simulink library "did"  (R2021b)
settings: Solver=VariableStepAuto  StartTime=0.0  StopTime=10.0  RelTol=1e-3
undefined symbols (not defined in the file): ADID_DODRange_pct, ADID_SOCRange_pct, ADID_TempRange_C, DiscIntNeverNeededParam, ENUM_CHRGPLUGSTA_AC, ENUM_CHRGPLUGSTA_DC, ENUM_CHRGPLUGSTA_NONE, ENUM_DRIVETRAIN_AWD, ENUM_DRIVETRAIN_FWD, ENUM_DRIVETRAIN_RWD, ENUM_EXTCHRGSTS_CHARGING, ENUM_OBCV2LSTA_WORKING, ENUM_PWRSTASW_READY, ENUM_VEHICLETYPE_D21, ENUM_VEHICLETYPE_D31F25, ENUM_VEHICLETYPE_D31HAWD, ENUM_VEHICLETYPE_D31HRWD, HOUR2SEC, HUNDRED, KDID_CPSAVehSpdThres_kph, KDID_DIDModelVersion_raw, KDID_DoDChrgCycle_s, KDID_FiveKmEquivEnergy_Wh, KDID_FlashInitDIDModelVersion_raw, KDID_IPSAVehSpdThres_kph, KDID_PropActiveTripThres_s, KDID_PSARResetThres_sec, KDID_RESSCNTSDODRNGAXIS_enum, KDID_RESSTIMESOCRNGAXIS_enum, KDID_RESSTTEMPRNGAXIS_enum, KDID_WarnUpPropActiveThres_s, KDID_WarnUpVehOperIdleThres_mph, KDID_WarnUpVehOperIdleThres_s, KDID_WarnUpVehOperThres_mph, KDID_WarnUpVehOperThres_s, KPH2MPH, KXX2XX, MINUSONE_FLOAT, ONE_FLOAT, ONE_INT, ONE_INT16, ONE_PERCENT, TRUE, UINT16_MAX, UINT32_MAX, XX2KXX, ZERO_FLOAT, ZERO_INT, ZERO_INT16, ZERO_INT32
libraries: hcu_lib x112, simulink x10, nmm x1
(part 2 of 4)

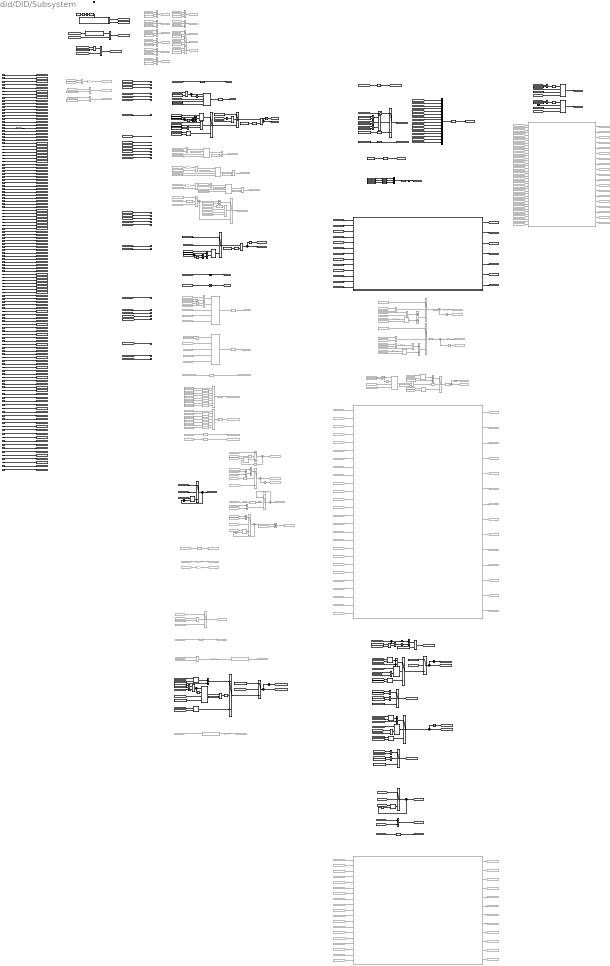
== system did/DID/Subsystem ==
  note: Flash data selector
  note: Model Version
  note: 0xF810: Protocol Identification
  note: 0xF896: Total Number of Propulsion System Active Events
  note: code_clear ??
  note: 0xF44D: Engine run time while MIL activated
  note: 0xF431: Distance traveled since DTCs cleared
  note: 0xF430: Number of warm-ups since DTCs cleared
  note: add debounce?
  note: 0xF421: Distance Traveled While MIL is Activated
  note: 0xF41F: Time Since Engine Start
  note: 0xF40D: Vehicle Speed Sensor
  note: 0xF449: Accelerator Pedal Position D
  note: 0xF44A: Accelerator Pedal Position E
  note: add debounce?
  note: 0xF44E: Engine run time since DTCs cleared
  note: 0xF45B: Hybrid Battery Pack Remaining Charge
  note: 0xF49A: Hybrid/EV Battery System Voltage
  note: 0xF4D1
  note: 0xF4DA
  note: 0xF4D4
  note: 0xF4B9
  note: 0xF4D6
  note: 0xF4D0
  note: SOH?
  note: 0xF4A6
  note: 0xF4B2
  note: Annex G
  note: Annex B
  note: 0xF802: Vehicle Identification Number
  note: 0xF804: Calibration Identifications
  note: 0xF813: Certification Test Group/Engine Family Number
  note: 0xF80A: ECUNAME
  note: 0xF881: High Voltage Battery Net Amp Hours
  note: 0xF882: Ignition Counter
  note: 0xF88C: Positive Kinetic Energy
  note: 0xF88D: Total Distance Travelled
  task_time_s : Inport
  VTQD_VehActSpd_kph : Inport  Port=2
  VPMM_SysPowerMode_enum : Inport  Port=3
  VPMM_DrivetrainSelect_enum : Inport  Port=4
  VDDM_VehMalfunLevel_enum : Inport  Port=5
  VDDM_LimpHomeAct_flg : Inport  Port=6
  VDDM_EnterNewOperCyc_flg : Inport  Port=7
  VINP_CANMsgValidESC1_flg : Inport  Port=8
  VINP_ODOMETER_km : Inport  Port=9
  VINP_CANMsgValidMETER1_flg : Inport  Port=10
  VINP_ClearDTCcmd_flg : Inport  Port=11
  VDHP_LowIdleAccPedal_flg : Inport  Port=12
  VDHP_EAPS1NRM_pct : Inport  Port=13
  VDHP_EAPS2NRM_pct : Inport  Port=14
  VINP_HVBattSOC_pct : Inport  Port=15
  VINP_HVBattPackVolt_V : Inport  Port=16
  VINP_ExtChrgSta_enum : Inport  Port=17
  VINP_HVBattCurr_A : Inport  Port=18
  VINP_HVBattVolt_V : Inport  Port=19
  VINP_ChrgPlugSta_enum : Inport  Port=20
  VINP_HVBPwrAvailChrg_kW : Inport  Port=21
  VINP_HVBCellVoltMax_mV : Inport  Port=22
  VINP_HVBCellVoltMin_mV : Inport  Port=23
  VINP_HVBSOH_pct : Inport  Port=24
  VINP_CANMsgValidMCUBR1_flg : Inport  Port=25
  VINP_CANMsgValidBMS6_flg : Inport  Port=26
  VINP_CANMsgValidBMS1_flg : Inport  Port=27
  VINP_CANMsgValidCCU2_flg : Inport  Port=28
  VINP_CANMsgValidBMS4_flg : Inport  Port=29
  VINP_CellTempAvg_C : Inport  Port=30
  VINP_OBCV2LSta_enum : Inport  Port=31
  VINP_RrMCUDCBusCurr_A : Inport  Port=32
  VINP_RrMCUDCBusVolt_V : Inport  Port=33
  VINP_FrMCUDCBusCurr_A : Inport  Port=34
  VINP_FrMCUDCBusVolt_V : Inport  Port=35
  VINP_CANMsgValidMCUBF1_flg : Inport  Port=36
  VINP_HVBMTempMax_C : Inport  Port=37
  VINP_HVBMTempMin_C : Inport  Port=38
  VINP_MCUBRRealPwrKwSta_kW : Inport  Port=39
  VINP_MCUBFRealPwrKwSta_kW : Inport  Port=40
  VINP_CANMsgValidBMS3_flg : Inport  Port=41
  VINP_VehicleType_enum : Inport  Port=42
  VINP_CarModel1_cnt : Inport  Port=43
  VINP_CarModel2_cnt : Inport  Port=44
  VINP_CarModel3_cnt : Inport  Port=45
  VINP_ECU1_cnt : Inport  Port=46
  VINP_ECU2_cnt : Inport  Port=47
  VINP_Major1_cnt : Inport  Port=48
  VINP_Major2_cnt : Inport  Port=49
  VINP_Minor1_cnt : Inport  Port=50
  VINP_Minor2_cnt : Inport  Port=51
  VINP_Patch1_cnt : Inport  Port=52
  VINP_Patch2_cnt : Inport  Port=53
  VINP_Country1_cnt : Inport  Port=54
  VINP_Country2_cnt : Inport  Port=55
  VINP_Variation_cnt : Inport  Port=56
  VINP_ECUGen1_cnt : Inport  Port=57
  VINP_ECUGen2_cnt : Inport  Port=58
  VINP_FlashMILDIST_km : Inport  Port=59
  VINP_FlashWARMUPS_cnt : Inport  Port=60
  VINP_FlashDelayCLRDIST_km : Inport  Port=61
  VINP_FlashMILTime_min : Inport  Port=62
  VINP_FlashCLRTime_min : Inport  Port=63
  VINP_FlashNUMPSATRIPSFLTMEMCLR_cnt : Inport  Port=64
  VINP_FlashPSAR_sec : Inport  Port=65
  VINP_FlashPSAL_sec : Inport  Port=66
  VINP_FlashIPSAR_sec : Inport  Port=67
  VINP_FlashIPSAL_sec : Inport  Port=68
  VINP_FlashCPSAR_sec : Inport  Port=69
  VINP_FlashCPSAL_sec : Inport  Port=70
  VINP_FlashHVBNAH_Ah : Inport  Port=71
  VINP_FlashIGNCNTR_cnt : Inport  Port=72
  VINP_FlashTNBCPSAR_Ahr : Inport  Port=73
  VINP_FlashTNBCPSAL_Ahr : Inport  Port=74
  VINP_FlashTNECPSAR_kWh : Inport  Port=75
  VINP_FlashTNECPSAL_kWh : Inport  Port=76
  VINP_FlashTEBPSAR_kWh : Inport  Port=77
  VINP_FlashTEBPSAL_kWh : Inport  Port=78
  VINP_FlashTGEOVCR_kWh : Inport  Port=79
  VINP_FlashTGEOVCL_kWh : Inport  Port=80
  VINP_FlashGECHGOVCDCR_kWh : Inport  Port=81
  VINP_FlashGECHGOVCDCL_kWh : Inport  Port=82
  VINP_FlashGECHGOVCACR_kWh : Inport  Port=83
  VINP_FlashGECHGOVCACL_kWh : Inport  Port=84
  VINP_FlashRESSV2XENNONPSAR_kWh : Inport  Port=85
  VINP_FlashRESSV2XENNONPSAL_kWh : Inport  Port=86
  VINP_FlashODOMETER_km : Inport  Port=87
  VINP_FlashPKERNumerator_kphsqr : Inport  Port=88
  VINP_FlashPKELNumerator_kphsqr : Inport  Port=89
  VINP_FlashResetCDEODTR_km : Inport  Port=90
  VINP_FlashTempPSAR_sec : Inport  Port=91
  VINP_FlashAvgBattTempPSAR_C : Inport  Port=92
  VINP_FlashTempPSAL_sec : Inport  Port=93
  VINP_FlashAvgBattTempPSAL_C : Inport  Port=94
  VINP_FlashOVCR_sec : Inport  Port=95
  VINP_FlashAvgBattTempOVCR_C : Inport  Port=96
  VINP_FlashOVCL_sec : Inport  Port=97
  VINP_FlashAvgBattTempOVCL_C : Inport  Port=98
  VINP_FlashOFFR_sec : Inport  Port=99
  VINP_FlashAvgBattTempOFFR_C : Inport  Port=100
  VINP_FlashOFFL_sec : Inport  Port=101
  VINP_FlashAvgBattTempOFFL_C : Inport  Port=102
  VINP_FlashHVBNE_kWh : Inport  Port=103
  VINP_FlashQTYPSATRIPSR_cnt : Inport  Port=104
  VINP_FlashQTYPSATRIPSL_cnt : Inport  Port=105
  VINP_FlashRESSCNTDODRNGR_cnt : Inport  Port=106
  VINP_FlashETMBTOER_kWh : Inport  Port=107
  VINP_FlashETMBTOEL_kWh : Inport  Port=108
  VINP_FlashRESSCNTDODRNGL_cnt : Inport  Port=109
  VINP_FlashETMATOER_kWh : Inport  Port=110
  VINP_FlashETMATOEL_kWh : Inport  Port=111
  VINP_FlashRESSTIMESOCPSARNGR_s : Inport  Port=112
  VINP_FlashRESSTIMESOCPSARNGL_s : Inport  Port=113
  VINP_FlashRESSTIMESOCCHGRNGR_s : Inport  Port=114
  VINP_FlashRESSTIMESOCOFFRNGL_s : Inport  Port=115
  VINP_FlashMAXBATTEMPL_C : Inport  Port=116
  VINP_FlashMINBATTEMPL_C : Inport  Port=117
  VINP_FlashRESSTIMESOCCHGRNGL_s : Inport  Port=118
  VINP_FlashRESSTIMESOCOFFRNGR_s : Inport  Port=119
  VINP_FlashAVGBATTEMPL_sec : Inport  Port=120
  VINP_FlashAVGBATTEMPL_C : Inport  Port=121
  VINP_VinCode_cnt : Inport  Port=122
  VINP_FlashModelVersion_raw : Inport  Port=123
  VINP_FlashModelVersionChksum_raw : Inport  Port=124
  Enable : EnablePort
  0xF819: Total Propulsion System Active Time : Subsystem
  0xF885 - 0xF88B : Subsystem  Commented=on
  0xF88E - 0xF890 : Subsystem  Commented=on
  0xF898-0xF8 : Subsystem  Commented=on
  1-D Lookup Table : Lookup_n-D  NumberOfTableDimensions=1  BreakpointsForDimension1=[ENUM_DRIVETRAIN_RWD;ENUM_DRIVETRAIN_FWD;ENUM_DRIVETRAIN_AWD]  Table=[uint8('R');uint8('F');uint8('A')]  InterpMethod=Nearest  InternalRulePriority=Speed  RndMeth=Simplest  InputSameDT=on
  AND : Logic  Commented=on  AllPortsSameDT=off  OutDataTypeStr=boolean
  AND2 : Logic  AllPortsSameDT=off  OutDataTypeStr=boolean
  AND6 : Logic  AllPortsSameDT=off  OutDataTypeStr=boolean
  Add : Sum
  Add1 : Sum  Commented=on
  Add2 : Sum
  Add3 : Sum
  Add6 : Sum  Commented=on
  Bitwise OR1 : simulink/Logic and Bit Operations/Bitwise Operator  Commented=on  logicop=OR  UseBitMask=off  NumInputPorts=7  BitMask=bin2dec('00000000000000000000')  BitMaskRealWorld=Stored Integer
  Bitwise OR123 : simulink/Logic and Bit Operations/Bitwise Operator  Commented=on  logicop=OR  UseBitMask=off  NumInputPorts=8  BitMask=bin2dec('00000000000000000000')  BitMaskRealWorld=Stored Integer
  Cast To Boolean : DataTypeConversion  OutDataTypeStr=boolean
  Checksum : Subsystem
  Constant{,5,26,28,34} (5 alike) : Constant  Value=ENUM_PWRSTASW_READY
  Constant1 : Constant  Value=UINT32_MAX
  Constant10 : Constant  Commented=on  Value=KDID_WarnUpVehOperThres_s
  Constant{32,59,65..68,105} (7 alike) : Constant  Commented=on  Value=ZERO_FLOAT
  Constant11 : Constant  Commented=on  Value=KDID_WarnUpVehOperThres_s
  Constant113 : Constant  Value=ZERO_FLOAT
  Constant12 : Constant  Commented=on  Value=KDID_WarnUpVehOperIdleThres_s
  Constant13 : Constant  Commented=on  Value=KDID_WarnUpVehOperIdleThres_s
  Constant14 : Constant  Commented=on  Value=KDID_WarnUpVehOperIdleThres_mph
  Constant{15,42,44..45,47..48,51..54,57..58,61..63,69..77} (24 alike) : Constant  Commented=on  Value=ZERO_INT
  Constant16 : Constant  Value=ZERO_FLOAT
  Constant17 : Constant  Value=UINT16_MAX
  Constant{6,18..19,25} (4 alike) : Constant  Commented=on  Value=ENUM_PWRSTASW_READY
  Constant2 : Constant  Commented=on  Value=ONE_INT
  Constant20 : Constant  Commented=on  Value=UINT16_MAX
  Constant21 : Constant  Value=ZERO_INT32
  Constant22 : Constant  Value=ONE_PERCENT  OutDataTypeStr=single
  Constant23 : Constant  Value=ZERO_INT16
  Constant24 : Constant  Commented=on  Value=UINT16_MAX
  Constant27 : Constant  Value=ONE_INT16
  Constant29 : Constant  Value=KDID_PropActiveTripThres_s
  Constant3 : Constant  Value=ZERO_FLOAT
  Constant30 : Constant  Value=KDID_PropActiveTripThres_s
  Constant31 : Constant  Commented=on  Value=ENUM_EXTCHRGSTS_CHARGING
  Constant33 : Constant  Value=UINT32_MAX
  Constant35 : Constant  Value=UINT32_MAX
  Constant36 : Constant  Value=ONE_INT
  Constant37 : Constant  Value=ZERO_FLOAT  OutDataTypeStr=uint16
  Constant38 : Constant  Commented=on  Value=KDID_PropActiveTripThres_s
  Constant39 : Constant  Value=ENUM_DRIVETRAIN_RWD
  Constant4 : Constant  Value=UINT16_MAX
  Constant40 : Constant  Value=ENUM_DRIVETRAIN_RWD
  Constant41 : Constant  Value=ENUM_DRIVETRAIN_RWD
  Constant43 : Constant  Commented=on  Value=ONE_INT
  Constant46 : Constant  Value=ONE_PERCENT  OutDataTypeStr=single
  Constant49 : Constant  Commented=on  Value=KDID_PropActiveTripThres_s
  Constant50 : Constant  Value=ZERO_FLOAT  OutDataTypeStr=single
  Constant55 : Constant  Value=KDID_FlashInitDIDModelVersion_raw
  Constant56 : Constant  Value=ZERO_FLOAT  OutDataTypeStr=single
  Constant60 : Constant  Value=ONE_FLOAT
  Constant64 : Constant  Value=TRUE
  Constant7 : Constant  Commented=on  Value=KDID_WarnUpPropActiveThres_s
  Constant79 : Constant  Commented=on  Value=ONE_INT16
  Constant8 : Constant  Commented=on  Value=KDID_WarnUpPropActiveThres_s
  Constant9 : Constant  Commented=on  Value=KDID_WarnUpVehOperThres_mph
  Data Type Conversion : DataTypeConversion  OutDataTypeStr=single
  Data Type Conversion1 : DataTypeConversion  OutDataTypeStr=uint16
  Data Type Conversion10 : DataTypeConversion  Commented=on  OutDataTypeStr=uint16
  Data Type Conversion{4..5,11,14} (4 alike) : DataTypeConversion  OutDataTypeStr=uint8
  Data Type Conversion{6..8,12,15} (5 alike) : DataTypeConversion  Commented=on
  Data Type Conversion13 : DataTypeConversion
  Data Type Conversion16 : DataTypeConversion  Commented=on  OutDataTypeStr=uint8
  Data Type Conversion17 : DataTypeConversion  Commented=on  OutDataTypeStr=uint8
  Data Type Conversion2 : DataTypeConversion  OutDataTypeStr=single
  Data Type Conversion23 : DataTypeConversion  Commented=on  OutDataTypeStr=single
  Data Type Conversion25 : DataTypeConversion  Commented=on  OutDataTypeStr=single
  Data Type Conversion29 : DataTypeConversion  Commented=on  OutDataTypeStr=uint16
  Data Type Conversion3 : DataTypeConversion  OutDataTypeStr=single
  Data Type Conversion9 : DataTypeConversion  Commented=on  OutDataTypeStr=uint16
  Delay : Delay  DelayLengthSource=Input port  DelayLengthUpperLimit=255
      settings: InputPortMap=u0,p1
  Delay1 : Delay
  Delay2 : Delay  Commented=on  DelayLength=1
  Detect Decrease : simulink/Logic and Bit Operations/Detect Decrease  Commented=on  vinit=0.0  OutDataTypeStr=boolean
  Detect Increase : simulink/Logic and Bit Operations/Detect Increase  vinit=0.0  OutDataTypeStr=boolean
  Detect Increase1 : simulink/Logic and Bit Operations/Detect Increase  vinit=0.0  OutDataTypeStr=boolean
  Detect Increase2 : simulink/Logic and Bit Operations/Detect Increase  Commented=on  vinit=0.0  OutDataTypeStr=boolean
  Detect Increase3 : simulink/Logic and Bit Operations/Detect Increase  vinit=0.0  OutDataTypeStr=boolean
  Detect Increase4 : simulink/Logic and Bit Operations/Detect Increase  Commented=on  vinit=0.0  OutDataTypeStr=boolean
  Detect Increase5 : simulink/Logic and Bit Operations/Detect Increase  Commented=on  vinit=0.0  OutDataTypeStr=boolean
  Divide : Product  Inputs=*/
  Divide1 : Product  Inputs=*/
  Divide2 : Product  Inputs=*/
  Equal{,2,9,13,15..17,21..22} (9 alike) : RelationalOperator  Operator===  OutDataTypeStr=boolean  RndMeth=Simplest
  Equal{1,8,10,12,18} (5 alike) : RelationalOperator  Commented=on  Operator===  OutDataTypeStr=boolean  RndMeth=Simplest
  Equal11 : RelationalOperator  OutDataTypeStr=boolean  RndMeth=Simplest
  Equal{3..5,7,14} (5 alike) : RelationalOperator  Commented=on  OutDataTypeStr=boolean  RndMeth=Simplest
  Equal19 : RelationalOperator  Operator=>  OutDataTypeStr=boolean  RndMeth=Simplest
  Equal20 : RelationalOperator  Operator=>  OutDataTypeStr=boolean  RndMeth=Simplest
  Equal23 : RelationalOperator  OutDataTypeStr=boolean  RndMeth=Simplest
  Equal6 : RelationalOperator  Commented=on  Operator=<=  OutDataTypeStr=boolean  RndMeth=Simplest
  From100 : From  Commented=on  GotoTag=VINP_FlashRESSV2XENNONPSAR_kWh
  From101 : From  Commented=on  GotoTag=VINP_FlashRESSV2XENNONPSAL_kWh
  From102 : From  Commented=on  GotoTag=VINP_CANMsgValidCCU2_flg
  From103 : From  Commented=on  GotoTag=VINP_ChrgPlugSta_enum
  From{15,17,20,31,35,75,106,158..159,162,246} (11 alike) : From  Commented=on  GotoTag=task_time_s
  From107 : From  Commented=on  GotoTag=VINP_CellTempAvg_C
  From108 : From  Commented=on  GotoTag=VINP_FlashTempPSAR_sec
  From110 : From  Commented=on  GotoTag=VDID_FlashAvgBattTempPSAR_C
  From111 : From  Commented=on  GotoTag=VINP_FlashTempPSAL_sec
  From112 : From  Commented=on  GotoTag=VDID_FlashAvgBattTempPSAL_C
  From113 : From  Commented=on  GotoTag=VINP_FlashOVCR_sec
  From116 : From  Commented=on  GotoTag=VDID_FlashAvgBattTempOVCR_C
  From117 : From  Commented=on  GotoTag=VINP_FlashOVCL_sec
  From125 : From  Commented=on  GotoTag=VDID_FlashAvgBattTempOVCL_C
  From129 : From  Commented=on  GotoTag=VINP_FlashOFFR_sec
  From131 : From  Commented=on  GotoTag=VDID_FlashAvgBattTempOFFR_C
  From132 : From  Commented=on  GotoTag=VINP_FlashOFFL_sec
  From133 : From  Commented=on  GotoTag=VDID_FlashAvgBattTempOFFL_C
  From{14,30,60,76,96,134,261} (7 alike) : From  Commented=on  GotoTag=VPMM_SysPowerMode_enum
  From135 : From  Commented=on  GotoTag=VDID_HVBattPwr_kW
  From136 : From  Commented=on  GotoTag=VINP_CANMsgValidBMS4_flg
  From140 : From  Commented=on  GotoTag=VINP_CANMsgValidBMS6_flg
  From141 : From  Commented=on  GotoTag=VDID_FlashHVBNAH_Ah
  From142 : From  Commented=on  GotoTag=VDID_NoteAResetCondition_flg
  From152 : From  Commented=on  GotoTag=VDID_DelayHVBNAH_As
  From153 : From  Commented=on  GotoTag=VINP_DIDResetNetAhrs_flg
  From{41,46,74,154,160,272,325} (7 alike) : From  Commented=on  GotoTag=VDID_HVBattCurr_A
  From155 : From  Commented=on  GotoTag=VINP_DIDResetNetAhrs_flg
  From{24,34,37..38,79,156..157,208} (8 alike) : From  Commented=on  GotoTag=VINP_ClearDTCcmd_flg
  From16 : From  Commented=on  GotoTag=VTQD_VehActSpd_kph
  From{40,48,161,273} (4 alike) : From  Commented=on  GotoTag=VINP_HVBattVolt_V
  From163 : From  Commented=on  GotoTag=VDID_FlashHVBNE_kWh
  From164 : From  Commented=on  GotoTag=VDID_DelayHVBNE_kWs
  From177 : From  Commented=on  GotoTag=VDID_DelayIGNCNTR_cnt
  From178 : From  Commented=on  GotoTag=VINP_FlashIGNCNTR_cnt
  From179 : From  Commented=on  GotoTag=VDID_DelayIGNCNTR_cnt
  From18 : From  Commented=on  GotoTag=VDHP_LowIdleAccPedal_flg
  From180 : From  Commented=on  GotoTag=VINP_FlashIGNCNTR_cnt
  From19 : From  Commented=on  GotoTag=VTQD_VehActSpd_kph
  From21 : From  Commented=on  GotoTag=KDID_WarnUpPropActive_flg
  From22 : From  Commented=on  GotoTag=KDID_WarnUpVehOper_flg
  From222 : From  Commented=on  GotoTag=VINP_OBCV2LSta_enum
  From23 : From  Commented=on  GotoTag=KDID_WarnUpVehOperIdle_flg
  From245 : From  Commented=on  GotoTag=VDID_HVBattPwr_kW
  From247 : From  Commented=on  GotoTag=VINP_CANMsgValidBMS1_flg
  From248 : From  Commented=on  GotoTag=VDID_NoteAResetCondition_flg
  From249 : From  Commented=on  GotoTag=VINP_FlashRESSCNTDODRNGR_cnt
  From250 : From  Commented=on  GotoTag=VINP_FlashRESSCNTDODRNGL_cnt
  From251 : From  Commented=on  GotoTag=VINP_RrMCUDCBusCurr_A
  From252 : From  Commented=on  GotoTag=VINP_RrMCUDCBusVolt_V
  From253 : From  Commented=on  GotoTag=VINP_FlashETMATOER_kWh
  From254 : From  Commented=on  GotoTag=VINP_FlashETMATOEL_kWh
  From255 : From  Commented=on  GotoTag=VINP_CANMsgValidMCUBR1_flg
  From256 : From  Commented=on  GotoTag=VINP_FrMCUDCBusCurr_A
  From257 : From  Commented=on  GotoTag=VINP_FrMCUDCBusVolt_V
  From258 : From  Commented=on  GotoTag=VINP_FlashETMBTOER_kWh
  From259 : From  Commented=on  GotoTag=VINP_FlashETMBTOEL_kWh
  From260 : From  Commented=on  GotoTag=VINP_CANMsgValidMCUBF1_flg
  From262 : From  Commented=on  GotoTag=VINP_ChrgPlugSta_enum
  From263 : From  Commented=on  GotoTag=VINP_CANMsgValidBMS6_flg
  From264 : From  Commented=on  GotoTag=VINP_HVBattSOC_pct
  From265 : From  Commented=on  GotoTag=VINP_FlashRESSTIMESOCPSARNGR_s
  From266 : From  Commented=on  GotoTag=VINP_FlashRESSTIMESOCPSARNGL_s
  From267 : From  Commented=on  GotoTag=VINP_ExtChrgSta_enum
  From268 : From  Commented=on  GotoTag=VINP_FlashRESSTIMESOCCHGRNGR_s
  From269 : From  Commented=on  GotoTag=VINP_FlashRESSTIMESOCCHGRNGL_s
  From270 : From  Commented=on  GotoTag=VINP_FlashRESSTIMESOCOFFRNGR_s
  From271 : From  Commented=on  GotoTag=VINP_FlashRESSTIMESOCOFFRNGL_s
  From274 : From  Commented=on  GotoTag=VDID_HVBattPwr_kW
  From275 : From  Commented=on  GotoTag=VDID_FlashMAXBATTEMPL_C
  From276 : From  Commented=on  GotoTag=VINP_HVBMTempMax_C
  From{277,370,375,379..380} (5 alike) : From  Commented=on  GotoTag=VINP_CANMsgValidMETER1_flg
  From278 : From  Commented=on  GotoTag=VDID_FlashMINBATTEMPL_C
  From279 : From  Commented=on  GotoTag=VINP_HVBMTempMin_C
  From280 : From  Commented=on  GotoTag=VINP_CANMsgValidBMS4_flg
  From281 : From  Commented=on  GotoTag=VINP_FlashAVGBATTEMPL_sec
  From282 : From  Commented=on  GotoTag=VDID_FlashAVGBATTEMPL_C
  From283 : From  Commented=on  GotoTag=VINP_CellTempAvg_C
  From285 : From  Commented=on  GotoTag=VDID_HVBattPwrDischrg_kW
  From286 : From  Commented=on  GotoTag=VINP_MCUBRRealPwrKwSta_kW
  From287 : From  Commented=on  GotoTag=VINP_MCUBFRealPwrKwSta_kW
  From288 : From  Commented=on  GotoTag=VINP_CANMsgValidBMS3_flg
  From3 : From  Commented=on  GotoTag=VDDM_EnterNewOperCyc_flg
  From32 : From  Commented=on  GotoTag=VDDM_LimpHomeActTmp_flg
  From33 : From  Commented=on  GotoTag=VDDM_LimpHomeAct_flg
  From{335,337,339..343,345,354..356} (11 alike) : From  Commented=on  GotoTag=VDID_FlashValid_flg
  From336 : From  Commented=on  GotoTag=VINP_FlashHVBNAH_Ah
  From338 : From  Commented=on  GotoTag=VINP_FlashHVBNE_kWh
  From344 : From  Commented=on  GotoTag=VINP_FlashAvgBattTempPSAL_C
  From346 : From  Commented=on  GotoTag=VINP_FlashAvgBattTempOVCR_C
  From347 : From  Commented=on  GotoTag=VINP_FlashAvgBattTempOVCL_C
  From348 : From  Commented=on  GotoTag=VINP_FlashAvgBattTempOFFR_C
  From349 : From  Commented=on  GotoTag=VINP_FlashAvgBattTempPSAR_C
  From350 : From  Commented=on  GotoTag=VINP_FlashAvgBattTempOFFL_C
  From351 : From  Commented=on  GotoTag=VINP_FlashMAXBATTEMPL_C
  From352 : From  Commented=on  GotoTag=VINP_FlashMINBATTEMPL_C
  From353 : From  Commented=on  GotoTag=VINP_FlashAVGBATTEMPL_C
  From{357,368,371,373,381} (5 alike) : From  Commented=on  GotoTag=VINP_ODOMETER_km
  From367 : From  Commented=on  GotoTag=VINP_FlashODOMETER_km
  From369 : From  Commented=on  GotoTag=VINP_FlashODOMETER_km
  From372 : From  Commented=on  GotoTag=VDID_ODOMETERLostConn_km
  From374 : From  Commented=on  GotoTag=VDID_ODOMETERLostDelay_km
  From376 : From  Commented=on  GotoTag=VDID_ODOMETERLostDelay_km
  From377 : From  Commented=on  GotoTag=VDID_ODOMETERLost_km
  From378 : From  Commented=on  GotoTag=VINP_FlashODOMETERLost_km
  From39 : From  Commented=on  GotoTag=VINP_HVBattSOC_pct
  From51 : From  Commented=on  GotoTag=VDID_HVBattPwrChrg_kW
  From52 : From  Commented=on  GotoTag=VINP_HVBPwrAvailChrg_kW
  From54 : From  Commented=on  GotoTag=VINP_HVBSOH_pct
  From55 : From  Commented=on  GotoTag=VINP_HVBCellVoltMax_mV
  From56 : From  Commented=on  GotoTag=VINP_HVBCellVoltMin_mV
  From61 : From  Commented=on  GotoTag=VINP_ExtChrgSta_enum
  From77 : From  Commented=on  GotoTag=VINP_FlashTNBCPSAR_Ahr
  From78 : From  Commented=on  GotoTag=VINP_FlashMILTime_min
  From8 : From  Commented=on  GotoTag=VINP_FlashWARMUPS_cnt
  From80 : From  Commented=on  GotoTag=VINP_FlashCLRTime_min
  From81 : From  Commented=on  GotoTag=VINP_CANMsgValidBMS1_flg
  From82 : From  Commented=on  GotoTag=VDID_NoteAResetCondition_flg
  From83 : From  Commented=on  GotoTag=VINP_FlashTNBCPSAL_Ahr
  From84 : From  Commented=on  GotoTag=VDID_HVBattPwrDischrg_kW
  From85 : From  Commented=on  GotoTag=VINP_FlashTNECPSAR_kWh
  From86 : From  Commented=on  GotoTag=VINP_FlashTNECPSAL_kWh
  From87 : From  Commented=on  GotoTag=VDID_HVBattPwrChrg_kW
  From88 : From  Commented=on  GotoTag=VINP_ChrgPlugSta_enum
  From89 : From  Commented=on  GotoTag=VINP_FlashTEBPSAR_kWh
  From90 : From  Commented=on  GotoTag=VINP_CANMsgValidBMS6_flg
  From91 : From  Commented=on  GotoTag=VINP_FlashTEBPSAL_kWh
  From92 : From  Commented=on  GotoTag=VINP_ExtChrgSta_enum
  From93 : From  Commented=on  GotoTag=VINP_FlashTGEOVCR_kWh
  From94 : From  Commented=on  GotoTag=VINP_FlashTGEOVCL_kWh
  From95 : From  Commented=on  GotoTag=VINP_FlashGECHGOVCDCR_kWh
  From97 : From  Commented=on  GotoTag=VINP_FlashGECHGOVCDCL_kWh
  From98 : From  Commented=on  GotoTag=VINP_FlashGECHGOVCACR_kWh
  From99 : From  Commented=on  GotoTag=VINP_FlashGECHGOVCACL_kWh
  Gain : Gain  Commented=on  Gain=KPH2MPH
  Gain1 : Gain  Commented=on  Gain=KPH2MPH
  Gain{2..3,14,20} (4 alike) : Gain  Commented=on  Gain=1/HOUR2SEC
  Gain19 : Gain  Gain=MINUSONE_FLOAT
  Gain21 : Gain  Commented=on  Gain=HOUR2SEC
  Gain{5..6,8,27} (4 alike) : Gain  Commented=on  Gain=XX2KXX
  Gain7 : Gain  Commented=on  Gain=HOUR2SEC
  Goto103 : Goto  Commented=on  GotoTag=VDID_HVBNE_kWh
  Goto12 : Goto  Commented=on  GotoTag=KDID_WarnUpPropActive_flg
  Goto13 : Goto  Commented=on  GotoTag=KDID_WarnUpVehOper_flg
  Goto135 : Goto  Commented=on  GotoTag=VDID_MILTIME_min
  Goto136 : Goto  Commented=on  GotoTag=VDID_CLRTIME_min
  Goto137 : Goto  Commented=on  GotoTag=VDID_BATSOC_pct
  Goto138 : Goto  Commented=on  GotoTag=VDID_HEVBATT_V
  Goto139 : Goto  Commented=on  GotoTag=VDID_IGNCNTR_cnt
  Goto14 : Goto  Commented=on  GotoTag=VDID_WARMUPS_cnt
  Goto140 : Goto  Commented=on  GotoTag=VDID_FlashHVBNAH_Ah
  Goto15 : Goto  Commented=on  GotoTag=KDID_WarnUpVehOperIdle_flg
  Goto153 : Goto  Commented=on  GotoTag=VDID_RESSCNTDODRNGR_cnt
  Goto154 : Goto  Commented=on  GotoTag=VDID_RESSCNTDODRNGL_cnt
  Goto155 : Goto  Commented=on  GotoTag=VDID_ETMATOER_kWh
  Goto156 : Goto  Commented=on  GotoTag=VDID_ETMATOEL_kWh
  Goto157 : Goto  Commented=on  GotoTag=VDID_ETMBTOER_kWh
  Goto158 : Goto  Commented=on  GotoTag=VDID_ETMBTOEL_kWh
  Goto159 : Goto  Commented=on  GotoTag=VDID_RESSTIMESOCPSARNGR_s
  Goto160 : Goto  Commented=on  GotoTag=VDID_RESSTIMESOCPSARNGL_s
  Goto161 : Goto  Commented=on  GotoTag=VDID_RESSTIMESOCCHGRNGR_s
  Goto162 : Goto  Commented=on  GotoTag=VDID_RESSTIMESOCCHGRNGL_s
  Goto163 : Goto  Commented=on  GotoTag=VDID_RESSTIMESOCOFFRNGR_s
  Goto164 : Goto  Commented=on  GotoTag=VDID_RESSTIMESOCOFFRNGL_s
  Goto165 : Goto  Commented=on  GotoTag=VDID_MAXBATTEMPL_C
  Goto166 : Goto  Commented=on  GotoTag=VDID_MINBATTEMPL_C
  Goto167 : Goto  Commented=on  GotoTag=VDID_AVGBATTEMPL_C
  Goto176 : Goto  Commented=on  GotoTag=VDID_RESSTTEMPRNGAXIS_enum
  Goto182 : Goto  Commented=on  GotoTag=VDID_RESSTIMESOCRNGAXIS_enum
  Goto183 : Goto  Commented=on  GotoTag=VDID_RESSCNTSDODRNGAXIS_enum
  Goto215 : Goto  Commented=on  GotoTag=VDID_AVGBATTEMPL_sec
  Goto216 : Goto  Commented=on  GotoTag=VDID_BattTempPSAR_sec
  Goto217 : Goto  Commented=on  GotoTag=VDID_BattTempPSAL_sec
  Goto218 : Goto  Commented=on  GotoTag=VDID_OVCR_sec
  Goto219 : Goto  Commented=on  GotoTag=VDID_OVCL_sec
  Goto22 : Goto  Commented=on  GotoTag=VDID_HVBattCurr_Ahps
  Goto220 : Goto  Commented=on  GotoTag=VDID_OFFR_sec
  Goto221 : Goto  Commented=on  GotoTag=VDID_OFFL_sec
  Goto227 : Goto  Commented=on  GotoTag=VDID_HVBATT_A
  Goto228 : Goto  Commented=on  GotoTag=VDID_HEVMODE_enum
  Goto229 : Goto  Commented=on  GotoTag=VDID_STASUP_enum
  Goto237 : Goto  Commented=on  GotoTag=VDID_FlashHVBNE_kWh
  Goto238 : Goto  Commented=on  GotoTag=VDID_FlashAvgBattTempPSAR_C
  Goto239 : Goto  Commented=on  GotoTag=VDID_FlashAvgBattTempPSAL_C
  Goto24 : Goto  Commented=on  GotoTag=VDID_HVESSENER_Whps
  Goto240 : Goto  Commented=on  GotoTag=VDID_FlashAvgBattTempOVCR_C
  Goto241 : Goto  Commented=on  GotoTag=VDID_FlashAvgBattTempOVCL_C
  Goto242 : Goto  Commented=on  GotoTag=VDID_FlashAvgBattTempOFFR_C
  Goto243 : Goto  Commented=on  GotoTag=VDID_FlashAvgBattTempOFFL_C
  Goto244 : Goto  Commented=on  GotoTag=VDID_FlashMAXBATTEMPL_C
  Goto245 : Goto  Commented=on  GotoTag=VDID_FlashMINBATTEMPL_C
  Goto246 : Goto  Commented=on  GotoTag=VDID_FlashAVGBATTEMPL_C
  Goto247 : Goto  Commented=on  GotoTag=VDID_ODOMETERLostConn_km
  Goto248 : Goto  Commented=on  GotoTag=VDID_ODOMETERLost_km
  Goto249 : Goto  Commented=on  GotoTag=VDID_ODOMETERLostDelay_km
  Goto25 : Goto  Commented=on  GotoTag=VDID_HVESSCHARGEACT_kW
  Goto250 : Goto  Commented=on  GotoTag=VDID_ODOMETER_km
  Goto251 : Goto  Commented=on  GotoTag=VINP_FlashODOMETERLost_km
  Goto26 : Goto  Commented=on  GotoTag=VDID_HVESSCHARGELIM_kW
  Goto27 : Goto  Commented=on  GotoTag=VDID_HVBCellVoltMax_V
  Goto29 : Goto  Commented=on  GotoTag=VDID_BATSOH_pct
  Goto30 : Goto  Commented=on  GotoTag=VDID_HVBCellVoltMin_V
  Goto50 : Goto  Commented=on  GotoTag=VDID_TNBCPSAR_Ahr
  Goto53 : Goto  Commented=on  GotoTag=VDID_TNBCPSAL_Ahr
  Goto54 : Goto  Commented=on  GotoTag=VDID_TNECPSAR_kWh
  Goto57 : Goto  Commented=on  GotoTag=VDID_TNECPSAL_kWh
  Goto58 : Goto  Commented=on  GotoTag=VDID_TEBPSAR_kWh
  Goto59 : Goto  Commented=on  GotoTag=VDID_TEBPSAL_kWh
  Goto60 : Goto  Commented=on  GotoTag=VDID_TGEOVCR_kWh
  Goto61 : Goto  Commented=on  GotoTag=VDID_TGEOVCL_kWh
  Goto62 : Goto  Commented=on  GotoTag=VDID_GECHGOVCDCR_kWh
  Goto63 : Goto  Commented=on  GotoTag=VDID_GECHGOVCDCL_kWh
  Goto64 : Goto  Commented=on  GotoTag=VDID_GECHGOVCACR_kWh
  Goto65 : Goto  Commented=on  GotoTag=VDID_GECHGOVCACL_kWh
  Goto66 : Goto  Commented=on  GotoTag=VDID_DelayIGNCNTR_cnt
  Goto67 : Goto  Commented=on  GotoTag=VDID_DelayHVBNAH_As
  Goto69 : Goto  Commented=on  GotoTag=VDID_DelayHVBNE_kWs
  Goto72 : Goto  Commented=on  GotoTag=VDID_RESSV2XENNONPSAR_kWh
  Goto73 : Goto  Commented=on  GotoTag=VDID_RESSV2XENNONPSAL_kWh
  Goto74 : Goto  Commented=on  GotoTag=VDID_AvgBattTempPSAR_C
  Goto75 : Goto  Commented=on  GotoTag=VDID_AvgBattTempPSAL_C
  Goto76 : Goto  Commented=on  GotoTag=VDID_AvgBattTempOVCR_C
  Goto77 : Goto  Commented=on  GotoTag=VDID_AvgBattTempOVCL_C
  Goto78 : Goto  Commented=on  GotoTag=VDID_AvgBattTempOFFR_C
  Goto79 : Goto  Commented=on  GotoTag=VDID_AvgBattTempOFFL_C
  Goto80 : Goto  Commented=on  GotoTag=VDID_HVBattPwr_kW
  Goto85 : Goto  Commented=on  GotoTag=VDID_HVBattPwrChrg_kW
  Goto86 : Goto  Commented=on  GotoTag=VDID_HVBattPwrDischrg_kW
  Goto99 : Goto  Commented=on  GotoTag=VDID_HVBNAH_Ahr
  Ground : Ground
  Initial Value{,1..6,34..37} (11 alike) : hcu_lib/Basic_Blocks/Initial Value
  Initial Value{7..12} (6 alike) : hcu_lib/Basic_Blocks/Initial Value  Commented=on
  Initializable_U32counter : hcu_lib/Basic_Blocks/Initializable_U32counter
  Initializable_U32counter1 : hcu_lib/Basic_Blocks/Initializable_U32counter
  Latch : hcu_lib/Basic_Blocks/Latch  Commented=on
  Latch1 : hcu_lib/Basic_Blocks/Latch  Commented=on
  Latch2 : hcu_lib/Basic_Blocks/Latch  Commented=on
  Logical Operator : Logic  Operator=OR  AllPortsSameDT=off  OutDataTypeStr=boolean
  Logical Operator1 : Logic  Inputs=3  AllPortsSameDT=off  OutDataTypeStr=boolean
  Logical Operator2 : Logic  Commented=on  Inputs=4  AllPortsSameDT=off  OutDataTypeStr=boolean
  Logical Operator3 : Logic  Commented=on  AllPortsSameDT=off  OutDataTypeStr=boolean
  Logical Operator4 : Logic  AllPortsSameDT=off  OutDataTypeStr=boolean
  Logical Operator5 : Logic  Commented=on  Operator=OR  AllPortsSameDT=off  OutDataTypeStr=boolean
  Logical Operator6 : Logic  Commented=on  Operator=OR  AllPortsSameDT=off  OutDataTypeStr=boolean
  Logical Operator7 : Logic  Commented=on  Operator=OR  AllPortsSameDT=off  OutDataTypeStr=boolean
  Logical Operator8 : Logic  Operator=NOT  AllPortsSameDT=off  OutDataTypeStr=boolean
  Logical Operator9 : Logic  AllPortsSameDT=off  OutDataTypeStr=boolean
  Max : MinMax  Inputs=2
  Max1 : MinMax  Inputs=2
  Max3 : MinMax  Function=max  Inputs=2
  Min14 : MinMax  Commented=on  Function=max  Inputs=2
  Min15 : MinMax  Commented=on  Inputs=2
  Minus : Sum  Inputs=+-
  Minus1 : Sum  Commented=on
  Minus2 : Sum  Commented=on
  Minus{3..6} (4 alike) : Sum  Commented=on  Inputs=+-
  Minus7 : Sum  Commented=on
  Minutes_Counter : hcu_lib/Basic_Blocks/Minutes_Counter  Commented=on
  Minutes_Counter1 : hcu_lib/Basic_Blocks/Minutes_Counter  Commented=on
  Mux : Mux  Inputs=3
  Mux1 : Mux  Inputs=16
  NOT{,1,3..4} (4 alike) : Logic  Operator=NOT  AllPortsSameDT=off  OutDataTypeStr=boolean
  NOT2 : Logic  Commented=on  Operator=NOT  AllPortsSameDT=off  OutDataTypeStr=boolean
  NOT6 : Logic  Commented=on  Operator=NOT  AllPortsSameDT=off  OutDataTypeStr=boolean
  OR : Logic  Operator=OR  Inputs=3  AllPortsSameDT=off  OutDataTypeStr=boolean
  Product{,1..2,4,27} (5 alike) : Product  Commented=on
  Reshape : Reshape
  Riemann Integral : hcu_lib/Basic_Blocks/Riemann Integral  Commented=on  Ts=0.005  Total_T=1
  Riemann Integral1 : hcu_lib/Basic_Blocks/Riemann Integral  Commented=on  Ts=0.005  Total_T=1
  Saturation : Saturate  UpperLimit=HUNDRED  LowerLimit=ZERO_FLOAT  OutDataTypeStr=single
  Saturation1 : Saturate  UpperLimit=HUNDRED  LowerLimit=ZERO_FLOAT  OutDataTypeStr=single
  Scheduler : Stateflow chart  TreatAsAtomicUnit=on
  Scheduler1 : Stateflow chart  TreatAsAtomicUnit=on
  Seconds_Counter : hcu_lib/Basic_Blocks/Seconds_Counter
  Shift Arithmetic1 : ArithShift  Commented=on  BitShiftNumber=4  BitShiftDirection=Left
  Shift Arithmetic10 : ArithShift  Commented=on  BitShiftNumber=3  BitShiftDirection=Left
  Shift Arithmetic11 : ArithShift  Commented=on  BitShiftNumber=7  BitShiftDirection=Left
  Shift Arithmetic2 : ArithShift  Commented=on  BitShiftNumber=5  BitShiftDirection=Left
  Shift Arithmetic3 : ArithShift  Commented=on  BitShiftNumber=6  BitShiftDirection=Left
  Shift Arithmetic311 : ArithShift  Commented=on  BitShiftNumber=1  BitShiftDirection=Left
  Shift Arithmetic312 : ArithShift  Commented=on  BitShiftNumber=2  BitShiftDirection=Left
  Shift Arithmetic313 : ArithShift  Commented=on  BitShiftNumber=3  BitShiftDirection=Left
  Shift Arithmetic4 : ArithShift  Commented=on  BitShiftNumber=7  BitShiftDirection=Left
  Shift Arithmetic5 : ArithShift  Commented=on  BitShiftNumber=4  BitShiftDirection=Left
  Shift Arithmetic6 : ArithShift  Commented=on  BitShiftNumber=5  BitShiftDirection=Left
  Shift Arithmetic7 : ArithShift  Commented=on  BitShiftNumber=6  BitShiftDirection=Left
  Shift Arithmetic8 : ArithShift  Commented=on  BitShiftNumber=1  BitShiftDirection=Left
  Square : Math  Operator=square  SaturateOnIntegerOverflow=on
  Square1 : Math  Operator=square  SaturateOnIntegerOverflow=on
  String Constant : StringConstant  String="\"EVCM\""
  String Constant1 : StringConstant  String="\"-\""
  String Constant2 : StringConstant  String="\"ElecVehicleCtrl\""
  String Constant3 : StringConstant  String="\"0\""
  String Constant4 : StringConstant  String="\"S\""
  String to ASCII : StringToASCII  OutputVectorSize=4
  String to ASCII1 : StringToASCII  OutputVectorSize=1
  String to ASCII2 : StringToASCII  OutputVectorSize=15
  String to ASCII3 : StringToASCII  OutputVectorSize=1
  String to ASCII4 : StringToASCII  OutputVectorSize=1
  Subsystem : Subsystem
  Subtract : Sum  Inputs=+-
  Subtract1 : Sum  Inputs=+-
  Subtract2 : Sum
  Subtract3 : Sum
  Subtract6 : Sum  Inputs=+-
  Switch{,1,4..7,9,11,16,61} (10 alike) : Switch  Criteria=u2 > Threshold
  Switch10 : Switch  Criteria=u2 ~= 0
      settings: AttributesFormatString=<%<Criteria>>
  Switch12 : Switch  Criteria=u2 ~= 0
      settings: AttributesFormatString=<%<Criteria>>
  Switch{2..3,8,13..15,17..31} (21 alike) : Switch  Commented=on  Criteria=u2 > Threshold
  Switch60 : Switch  Criteria=u2 ~= 0
      settings: AttributesFormatString=<%<Criteria>>
  Timer{1..3,5} (4 alike) : hcu_lib/Basic_Blocks/Timer  Commented=on
  Timer6 : hcu_lib/Basic_Blocks/Timer
  Unit Delay{,1..2,4..7,11,23} (9 alike) : UnitDelay  SampleTime=-1  HasFrameUpgradeWarning=on
  Unit Delay{3,8..10,13..14,20} (7 alike) : UnitDelay  Commented=on  SampleTime=-1  HasFrameUpgradeWarning=on
  VDID_VSS_kph : Outport
  VDID_RUNTM_s : Outport  Port=2
  VDID_MILDIST_km : Outport  Port=3
  VDID_CLRDIST_km : Outport  Port=4
  VDID_APPD_pct : Outport  Port=5
  VDID_APPE_pct : Outport  Port=6
  VDID_ODOMETER_km : Outport  Port=7
  VDID_NUMPSATRIPSFLTMEMCLR_cnt : Outport  Port=8
  VDID_PSAR_sec : Outport  Port=9
  VDID_PSAL_sec : Outport  Port=10
  VDID_IPSAR_sec : Outport  Port=11
  VDID_IPSAL_sec : Outport  Port=12
  VDID_CPSAR_sec : Outport  Port=13
  VDID_CPSAL_sec : Outport  Port=14
  VDID_PKER_kphsqr : Outport  Port=15
  VDID_PKEL_kphsqr : Outport  Port=16
  VDID_ResetCDEODTR_km : Outport  Port=17
  VDID_CDEODTR_km : Outport  Port=18
  VDID_CDEODTL_km : Outport  Port=19
  VDID_QTYPSATRIPSR_cnt : Outport  Port=20
  VDID_QTYPSATRIPSL_cnt : Outport  Port=21
  VDID_PRO TOCOLID_enum : Outport  Port=22
  VDID_CALID_cnt : Outport  Port=23
  VDID_ECUNAME_cnt : Outport  Port=24
  VDID_PKERNumerator_kphsqr : Outport  Port=25
  VDID_PKELNumerator_kphsqr : Outport  Port=26
  VDID_VinCode_cnt : Outport  Port=27
  VDID_DIDModelVersion_raw : Outport  Port=28
  VDID_DIDModelVersionChksum_raw : Outport  Port=29
  wires:
  task_time_s/1 -> [task_time_s]
  VTQD_VehActSpd_kph/1 -> [VTQD_VehActSpd_kph]
  [VTQD_VehActSpd_kph] -> Data Type Conversion/1
  Data Type Conversion/1 -> [VDID_VSS_kph]
  VPMM_SysPowerMode_enum/1 -> [VPMM_SysPowerMode_enum]
  [VPMM_SysPowerMode_enum] -> Equal/1
  Constant/1 -> Equal/2
  Equal/1 -> NOT1/1, Seconds_Counter/1
  NOT1/1 -> Seconds_Counter/2
  [task_time_s] -> Seconds_Counter/3
  Constant1/1 -> Seconds_Counter/4
  Seconds_Counter/1 -> Data Type Conversion1/1
  Data Type Conversion1/1 -> [VDID_RUNTM_s]
  VDDM_VehMalfunLevel_enum/1 -> [VDDM_VehMalfunLevel_enum]
  VINP_ODOMETER_km/1 -> [VINP_ODOMETER_km]
  Unit Delay1/1 -> Subtract/2
  Subtract/1 -> Add/2
  Unit Delay/1 -> [VDID_DelayMILDIST_km]
  Switch/1 -> Switch1/3
  VINP_ClearDTCcmd_flg/1 -> [VINP_ClearDTCcmd_flg]
  [VDDM_LimpHomeAct_flg] -> NOT/1
  NOT/1 -> Logical Operator/1
  [VINP_ClearDTCcmd_flg] -> Logical Operator/2
  Constant3/1 -> Switch1/1
  Switch1/1 -> Max/1
  Max/1 -> Unit Delay/1, [VDID_MILDIST_km]
  VINP_CANMsgValidMETER1_flg/1 -> [VINP_CANMsgValidMETER1_flg]
  [VDDM_LimpHomeAct_flg] -> Logical Operator1/1
  Logical Operator1/1 -> Switch/2
  [VDID_ODOMETER_km] -> Unit Delay1/1, Subtract/1
  Constant5/1 -> Equal2/2
  [VPMM_SysPowerMode_enum] -> Equal2/1
  Equal2/1 -> Logical Operator1/3
  VDDM_LimpHomeAct_flg/1 -> [VDDM_LimpHomeAct_flg]
  Logical Operator/1 -> Switch1/2
  VDDM_EnterNewOperCyc_flg/1 -> [VDDM_EnterNewOperCyc_flg]
  From3/1 -> Latch/1
  Latch/1 -> Logical Operator2/1
  Switch3/1 -> Add1/1, Switch2/3
  Constant2/1 -> Add1/2
  Add1/1 -> Switch2/1
  Constant6/1 -> Equal1/2
  Constant7/1 -> Timer1/4
  Equal1/1 -> Timer1/1
  From15/1 -> Timer1/3
  From14/1 -> Equal1/1
  Timer1/1 -> Equal3/1
  Constant8/1 -> Equal3/2
  From16/1 -> Gain/1
  Gain/1 -> Equal4/1
  Constant9/1 -> Equal4/2
  Equal4/1 -> Timer2/1
  From17/1 -> Timer2/3
  Constant10/1 -> Timer2/4
  Constant11/1 -> Equal5/2
  Timer2/1 -> Equal5/1
  VDHP_LowIdleAccPedal_flg/1 -> [VDHP_LowIdleAccPedal_flg]
  Timer3/1 -> Equal7/1
  Constant13/1 -> Equal7/2
  Constant12/1 -> Timer3/4
  From20/1 -> Timer3/3
  From34/1 -> Timer3/2
  Constant14/1 -> Equal6/2
  Gain1/1 -> Equal6/1
  From19/1 -> Gain1/1
  From18/1 -> AND/1
  AND/1 -> Timer3/1
  Equal6/1 -> AND/2
  Equal3/1 -> Goto12/1
  Equal5/1 -> Goto13/1
  Equal7/1 -> Goto15/1
  From21/1 -> Logical Operator2/2
  From22/1 -> Logical Operator2/3
  From23/1 -> Logical Operator2/4
  Logical Operator2/1 -> Switch2/2
  From8/1 -> Switch3/3
  From24/1 -> Latch1/1
  Constant15/1 -> Switch3/1
  Switch2/1 -> Goto14/1
  Latch1/1 -> Switch3/2
  [VINP_ClearDTCcmd_flg] -> Switch4/2
  [VDID_ODOMETER_km] -> Unit Delay2/1, Subtract1/1
  Unit Delay2/1 -> Subtract1/2
  Constant16/1 -> Switch4/1
  Switch4/1 -> Max1/1
  Unit Delay4/1 -> [VDID_DelayCLRDIST_km]
  VDHP_EAPS1NRM_pct/1 -> [VDHP_EAPS1NRM_pct]
  VDHP_EAPS2NRM_pct/1 -> [VDHP_EAPS2NRM_pct]
  [VDHP_EAPS1NRM_pct] -> Saturation/1
  [VDHP_EAPS2NRM_pct] -> Saturation1/1
  Saturation1/1 -> [VDID_APPE_pct]
  From30/1 -> Equal8/1
  Constant19/1 -> Equal8/2
  Equal8/1 -> Logical Operator3/2
  From32/1 -> Logical Operator3/1
  From33/1 -> NOT2/1
  From37/1 -> Timer2/2
  From38/1 -> Timer1/2
  VINP_HVBattSOC_pct/1 -> [VINP_HVBattSOC_pct]
  From39/1 -> Data Type Conversion6/1
  Data Type Conversion6/1 -> Goto137/1  "VDID_BATSOC_pct"
  VINP_HVBattPackVolt_V/1 -> [VINP_HVBattPackVolt_V]
  From40/1 -> Data Type Conversion7/1
  [VINP_ODOMETER_km] -> Switch9/1
  Gain3/1 -> Riemann Integral1/1
  Switch9/1 -> Unit Delay5/1, [VDID_ODOMETER_km]
  Gain6/1 -> Goto27/1
  From51/1 -> Data Type Conversion12/1
  Data Type Conversion8/1 -> Goto29/1
  From54/1 -> Data Type Conversion8/1
  Equal10/1 -> Switch8/2
  From55/1 -> Gain6/1
  Switch8/1 -> Goto26/1
  From52/1 -> Switch8/1
  Constant31/1 -> Equal10/2
  From48/1 -> Product2/2
  Product2/1 -> Gain3/1  "VDID_HVBattPwr_W"
  Riemann Integral1/1 -> Goto24/1
  Equal11/1 -> Detect Increase/1
  Constant32/1 -> Switch8/3
  Constant29/1 -> Timer6/4
  Detect Increase/1 -> Switch6/2
  [task_time_s] -> Timer6/3
  Timer6/1 -> Equal11/1
  [VINP_ClearDTCcmd_flg] -> Switch5/2
  Gain5/1 -> Goto30/1
  From56/1 -> Gain5/1
  From61/1 -> Equal10/1
  Constant30/1 -> Equal11/2
  Constant27/1 -> Add3/2
  Add3/1 -> Switch6/1
  Riemann Integral/1 -> Gain2/1
  Constant23/1 -> Switch5/1
  [VINP_CANMsgValidMETER1_flg] -> Switch9/2
  [VPMM_SysPowerMode_enum] -> Equal9/1
  Constant28/1 -> Equal9/2
  [VDID_DelayMILDIST_km] -> Initial Value1/2
  [VINP_FlashMILDIST_km] -> Initial Value1/1
  Initial Value1/1 -> Switch/3
  [VINP_FlashMILDIST_km] -> Initial Value2/1
  [VDID_DelayMILDIST_km] -> Add/1
  Data Type Conversion9/1 -> Goto135/1
  Data Type Conversion10/1 -> Goto136/1
  Minutes_Counter1/1 -> Data Type Conversion10/1
  Constant18/1 -> Equal12/2
  From60/1 -> Equal12/1
  Equal12/1 -> Minutes_Counter1/1
  Logical Operator3/1 -> Minutes_Counter/1
  From31/1 -> Minutes_Counter/3
  Constant20/1 -> Minutes_Counter/4
  Minutes_Counter/1 -> Data Type Conversion9/1
  From35/1 -> Minutes_Counter1/3
  Constant24/1 -> Minutes_Counter1/4
  From79/1 -> Minutes_Counter1/2
  From46/1 -> Product2/1
  [VINP_ClearDTCcmd_flg] -> NOT3/1
  From41/1 -> Riemann Integral/1
  Gain2/1 -> Goto22/1
  VINP_ExtChrgSta_enum/1 -> [VINP_ExtChrgSta_enum]
  VINP_HVBattVolt_V/1 -> [VINP_HVBattVolt_V]
  VINP_ChrgPlugSta_enum/1 -> [VINP_ChrgPlugSta_enum]
  VINP_HVBPwrAvailChrg_kW/1 -> [VINP_HVBPwrAvailChrg_kW]
  VINP_HVBCellVoltMax_mV/1 -> [VINP_HVBCellVoltMax_mV]
  VINP_HVBCellVoltMin_mV/1 -> [VINP_HVBCellVoltMin_mV]
  VINP_HVBSOH_pct/1 -> [VINP_HVBSOH_pct]
  VINP_CANMsgValidMCUBR1_flg/1 -> [VINP_CANMsgValidMCUBR1_flg]
  VINP_CANMsgValidESC1_flg/1 -> [VINP_CANMsgValidESC1_flg]
  Switch13/1 -> Data Type Conversion23/1
  Product1/1 -> Minus2/1
  From155/1 -> Logical Operator6/1
  Product/1 -> Minus1/1
  Constant66/1 -> Switch21/1
  Data Type Conversion23/1 -> Gain20/1, Unit Delay13/1
  Switch21/1 -> Data Type Conversion25/1
  Minus2/1 -> Switch21/3
  Constant67/1 -> Switch13/1
  From153/1 -> Logical Operator5/1
  Minus1/1 -> Switch13/3
  From161/1 -> Product4/2
  From159/1 -> Product/2
  From157/1 -> Logical Operator5/2
  From158/1 -> Product1/2
  Logical Operator6/1 -> Switch13/2
  From156/1 -> Logical Operator6/2
  Logical Operator5/1 -> Switch21/2
  From160/1 -> Product4/1
  Initial Value11/1 -> Switch22/3
  From177/1 -> Initial Value11/2
  Detect Increase2/1 -> Switch22/2
  From179/1 -> Initial Value12/2
  Unit Delay20/1 -> Goto66/1
  From178/1 -> Initial Value11/1
  Switch22/1 -> Data Type Conversion29/1
  Initial Value12/1 -> Add6/1
  Add6/1 -> Switch22/1
  Constant79/1 -> Add6/2
  Data Type Conversion29/1 -> Goto139/1, Unit Delay20/1
  From180/1 -> Initial Value12/1
  Gain19/1 -> [VDID_HVBattCurr_A]
  Unit Delay13/1 -> Goto67/1
  From141/1 -> Gain7/1
  From152/1 -> Initial Value7/2
  Initial Value7/1 -> Minus1/2
  From164/1 -> Initial Value8/2
  From163/1 -> Gain21/1
  Initial Value8/1 -> Minus2/2
  Unit Delay14/1 -> Goto69/1
  Data Type Conversion25/1 -> Unit Delay14/1, Gain14/1
  Gain21/1 -> Initial Value8/1
  VINP_HVBattCurr_A/1 -> Gain19/1
  From154/1 -> Product/1
  Gain7/1 -> Initial Value7/1
  Product4/1 -> Gain8/1
  Gain8/1 -> Product1/1  "VDID_HVBattPwr_kW"
  NOT6/1 -> Timer5/2
  Constant25/1 -> Equal18/2
  Equal14/1 -> Detect Increase2/1
  From96/1 -> Equal18/1
  Timer5/1 -> Equal14/1
  Constant49/1 -> Equal14/2
  From162/1 -> Timer5/3
  Constant38/1 -> Timer5/4
  Equal18/1 -> NOT6/1, Timer5/1
  From78/1 -> Minutes_Counter/5
  From80/1 -> Minutes_Counter1/5
  Constant105/1 -> Min15/2
  From274/1 -> Min15/1
  Min15/1 -> Goto86/1
  Min14/1 -> Goto85/1
  From135/1 -> Min14/1
  Constant59/1 -> Min14/2
  Gain27/1 -> Goto80/1  "VDID_HVBattPwr_kW"
  Product27/1 -> Gain27/1
  From272/1 -> Product27/1
  From273/1 -> Product27/2
  Minus/1 -> Max3/1
  Unit Delay23/1 -> [VDID_DelayPKELNumerator_kphsqr]
  [VDID_PKENumeratorOneSec_kphsqr] -> Subtract3/2
  [VINP_FlashPKELNumerator_kphsqr] -> Initial Value37/1
  [VDID_NoteAResetCondition_flg] -> Switch61/2
  [VINP_CANMsgValidMCUBR1_flg] -> AND2/2
  Constant37/1 -> Switch11/3
  Constant113/1 -> Max3/2
  [task_time_s] -> Scheduler1/1(task_time_s)
  [VINP_CANMsgValidESC1_flg] -> AND6/1
  Divide1/1 -> Switch11/1
  Initial Value3/1 -> Switch61/3
  Subtract6/1 -> [VDID_CDEODTR_km]
  [VDID_ResetCDEODTR_km] -> Subtract6/2
  [VDID_ODOMETER_km] -> Data Type Conversion13/1
  [task_time_s] -> Scheduler/1(task_time_s)
  [VDID_ODOMETER_km] -> Subtract6/1
  Scheduler/1(trig_1sec) -> Switch60/2
  Constant22/1 -> Equal19/2
  Switch16/1 -> [VDID_PKEL_kphsqr]
  [VDID_CDEODTR_km] -> Divide1/2
  [VDID_ODOMETER_km] -> Switch61/1
  [VINP_FlashResetCDEODTR_km] -> Initial Value3/1
  Switch61/1 -> Unit Delay6/1, [VDID_ResetCDEODTR_km]
  Switch10/1 -> [VDID_PKERNumerator_kphsqr], Unit Delay11/1
  Switch60/1 -> Switch10/3
  AND2/1 -> Scheduler1/2(trigger)
  [VDID_NoteAResetCondition_flg] -> Switch10/2
  Initial Value36/1 -> Switch12/3
  [VDID_PKELNumerator_kphsqr] -> Divide2/1
  Unit Delay6/1 -> Initial Value3/2
  [VDID_CDEODTL_km] -> Equal20/1
  [task_time_s] -> Divide/2
  [VINP_FlashPKERNumerator_kphsqr] -> Initial Value35/1
  [VDID_PKERNumerator_kphsqr] -> Divide1/1
  Divide2/1 -> Switch16/1
  Delay/1 -> Square1/1
  Initial Value35/1 -> Subtract2/1
  Unit Delay11/1 -> [VDID_DelayPKERNumerator_kphsqr]
  [VINP_CANMsgValidMCUBR1_flg] -> AND6/2
  Constant60/1 -> Divide/1
  [VDID_PKENumeratorOneSec_kphsqr] -> Subtract2/2
  [VTQD_VehActSpd_kph] -> Square/1, Delay/1
  [VDID_DelayPKELNumerator_kphsqr] -> Initial Value36/2
  [VDID_DelayPKELNumerator_kphsqr] -> Initial Value37/2
  [VDID_DelayPKERNumerator_kphsqr] -> Initial Value35/2
  Square/1 -> Minus/1
  Divide/1 -> Delay/2
  Square1/1 -> Minus/2
  [VINP_FlashPKERNumerator_kphsqr] -> Initial Value34/1
  Switch12/1 -> Unit Delay23/1, [VDID_PKELNumerator_kphsqr]
  Equal19/1 -> Switch11/2
  Subtract3/1 -> Switch12/1
  [VINP_FlashPKELNumerator_kphsqr] -> Initial Value36/1
  Max3/1 -> [VDID_PKENumeratorOneSec_kphsqr]
  Subtract2/1 -> Switch60/1
  [VINP_CANMsgValidESC1_flg] -> AND2/1
  Constant56/1 -> Switch10/1
  [VDID_DelayPKERNumerator_kphsqr] -> Initial Value34/2
  Constant46/1 -> Equal20/2
  Constant50/1 -> Switch16/3
  Switch11/1 -> [VDID_PKER_kphsqr]
  [VDID_CDEODTR_km] -> Equal19/1
  AND6/1 -> Scheduler/2(trigger)
  [VDID_CDEODTL_km] -> Divide2/2
  Initial Value37/1 -> Subtract3/1
  Scheduler1/1(trig_1sec) -> Switch12/2
  Equal20/1 -> Switch16/2
  Initial Value34/1 -> Switch60/3
  Constant21/1 -> Seconds_Counter/5
  Data Type Conversion12/1 -> Goto25/1
  [VTQD_VehActSpd_kph] -> 0xF819: Total Propulsion System Active Time/5(VTQD_VehActSpd_kph)
  [VINP_CANMsgValidESC1_flg] -> 0xF819: Total Propulsion System Active Time/6(VINP_CANMsgValidESC1_flg)
  [VINP_CANMsgValidMCUBR1_flg] -> 0xF819: Total Propulsion System Active Time/7(VINP_CANMsgValidMCUBR1_flg)
  [VDHP_LowIdleAccPedal_flg] -> 0xF819: Total Propulsion System Active Time/4(VDHP_LowIdleAccPedal_flg)
  [VINP_FlashPSAR_sec] -> 0xF819: Total Propulsion System Active Time/8(VINP_FlashPSAR_sec)
  [VINP_ClearDTCcmd_flg] -> 0xF819: Total Propulsion System Active Time/3(VINP_ClearDTCcmd_flg)
  [VINP_FlashPSAL_sec] -> 0xF819: Total Propulsion System Active Time/9(VINP_FlashPSAL_sec)
  [task_time_s] -> 0xF819: Total Propulsion System Active Time/2(task_time_s)
  [VPMM_SysPowerMode_enum] -> 0xF819: Total Propulsion System Active Time/1(VPMM_SysPowerMode_enum)
  [VINP_FlashIPSAR_sec] -> 0xF819: Total Propulsion System Active Time/10(VINP_FlashIPSAR_sec)
  [VINP_FlashIPSAL_sec] -> 0xF819: Total Propulsion System Active Time/11(VINP_FlashIPSAL_sec)
  [VINP_FlashCPSAR_sec] -> 0xF819: Total Propulsion System Active Time/12(VINP_FlashCPSAR_sec)
  [VINP_FlashCPSAL_sec] -> 0xF819: Total Propulsion System Active Time/13(VINP_FlashCPSAL_sec)
  0xF819: Total Propulsion System Active Time/5(VDID_IPSAL_sec) -> [VDID_IPSAL_sec]
  0xF819: Total Propulsion System Active Time/6(VDID_CPSAR_sec) -> [VDID_CPSAR_sec]
  0xF819: Total Propulsion System Active Time/4(VDID_IPSAR_sec) -> [VDID_IPSAR_sec]
  0xF819: Total Propulsion System Active Time/7(VDID_CPSAL_sec) -> [VDID_CPSAL_sec]
  0xF819: Total Propulsion System Active Time/3(VDID_PSAL_sec) -> [VDID_PSAL_sec]
  0xF819: Total Propulsion System Active Time/2(VDID_PSAR_sec) -> [VDID_PSAR_sec]
  0xF819: Total Propulsion System Active Time/1(VDID_NoteAResetCondition_flg) -> [VDID_NoteAResetCondition_flg]
  From86/1 -> 0xF885 - 0xF88B/10(VINP_FlashTNECPSAL_kWh)
  From85/1 -> 0xF885 - 0xF88B/9(VINP_FlashTNECPSAR_kWh)
  From87/1 -> 0xF885 - 0xF88B/11(VDID_HVBattPwrChrg_kW)
  From84/1 -> 0xF885 - 0xF88B/8(VDID_HVBattPwrDischrg_kW)
  From88/1 -> 0xF885 - 0xF88B/12(VINP_ChrgPlugSta_enum)
  From83/1 -> 0xF885 - 0xF88B/7(VINP_FlashTNBCPSAL_Ahr)
  From89/1 -> 0xF885 - 0xF88B/13(VINP_FlashTEBPSAR_kWh)
  From82/1 -> 0xF885 - 0xF88B/6(VDID_NoteAResetCondition_flg)
  From81/1 -> 0xF885 - 0xF88B/5(VINP_CANMsgValidBMS1_flg)
  From90/1 -> 0xF885 - 0xF88B/14(VINP_CANMsgValidBMS6_flg)
  From77/1 -> 0xF885 - 0xF88B/4(VINP_FlashTNBCPSAR_Ahr)
  From91/1 -> 0xF885 - 0xF88B/15(VINP_FlashTEBPSAL_kWh)
  From76/1 -> 0xF885 - 0xF88B/3(VPMM_SysPowerMode_enum)
  From92/1 -> 0xF885 - 0xF88B/16(VINP_ExtChrgSta_enum)
  From75/1 -> 0xF885 - 0xF88B/2(task_time_s)
  From93/1 -> 0xF885 - 0xF88B/17(VINP_FlashTGEOVCR_kWh)
  From74/1 -> 0xF885 - 0xF88B/1(VDID_HVBattCurr_A)
  From94/1 -> 0xF885 - 0xF88B/18(VINP_FlashTGEOVCL_kWh)
  From95/1 -> 0xF885 - 0xF88B/19(VINP_FlashGECHGOVCDCR_kWh)
  From97/1 -> 0xF885 - 0xF88B/20(VINP_FlashGECHGOVCDCL_kWh)
  From98/1 -> 0xF885 - 0xF88B/21(VINP_FlashGECHGOVCACR_kWh)
  From99/1 -> 0xF885 - 0xF88B/22(VINP_FlashGECHGOVCACL_kWh)
  From100/1 -> 0xF885 - 0xF88B/23(VINP_FlashRESSV2XENNONPSAR_kWh)
  From101/1 -> 0xF885 - 0xF88B/24(VINP_FlashRESSV2XENNONPSAL_kWh)
  From102/1 -> 0xF885 - 0xF88B/25(VINP_CANMsgValidCCU2_flg)
  0xF885 - 0xF88B/4(VDID_TNECPSAL_kWh) -> Goto57/1
  0xF885 - 0xF88B/5(VDID_TEBPSAR_kWh) -> Goto58/1
  0xF885 - 0xF88B/3(VDID_TNECPSAR_kWh) -> Goto54/1
  0xF885 - 0xF88B/6(VDID_TEBPSAL_kWh) -> Goto59/1
  0xF885 - 0xF88B/2(VDID_TNBCPSAL_Ahr) -> Goto53/1
  0xF885 - 0xF88B/7(VDID_TGEOVCR_kWh) -> Goto60/1
  0xF885 - 0xF88B/1(VDID_TNBCPSAR_Ahr) -> Goto50/1
  0xF885 - 0xF88B/8(VDID_TGEOVCL_kWh) -> Goto61/1
  0xF885 - 0xF88B/9(VDID_GECHGOVCDCR_kWh) -> Goto62/1
  0xF885 - 0xF88B/10(VDID_GECHGOVCDCL_kWh) -> Goto63/1
  0xF885 - 0xF88B/11(VDID_GECHGOVCACR_kWh) -> Goto64/1
  0xF885 - 0xF88B/12(VDID_GECHGOVCACL_kWh) -> Goto65/1
  0xF885 - 0xF88B/13(VDID_RESSV2XENNONPSAR_kWh) -> Goto72/1
  0xF885 - 0xF88B/14(VDID_RESSV2XENNONPSAL_kWh) -> Goto73/1
  From107/1 -> 0xF88E - 0xF890/7(VINP_CellTempAvg_C)
  From106/1 -> 0xF88E - 0xF890/6(task_time_s)
  From108/1 -> 0xF88E - 0xF890/8(VINP_FlashTempPSAR_sec)
  From103/1 -> 0xF88E - 0xF890/5(VINP_ChrgPlugSta_enum)
  From110/1 -> 0xF88E - 0xF890/9(VDID_FlashAvgBattTempPSAR_C)
  From111/1 -> 0xF88E - 0xF890/10(VINP_FlashTempPSAL_sec)
  From142/1 -> 0xF88E - 0xF890/4(VDID_NoteAResetCondition_flg)
  From140/1 -> 0xF88E - 0xF890/3(VINP_CANMsgValidBMS6_flg)
  From112/1 -> 0xF88E - 0xF890/11(VDID_FlashAvgBattTempPSAL_C)
  From113/1 -> 0xF88E - 0xF890/12(VINP_FlashOVCR_sec)
  From136/1 -> 0xF88E - 0xF890/2(VINP_CANMsgValidBMS4_flg)
  From134/1 -> 0xF88E - 0xF890/1(VPMM_SysPowerMode_enum)
  From116/1 -> 0xF88E - 0xF890/13(VDID_FlashAvgBattTempOVCR_C)
  From117/1 -> 0xF88E - 0xF890/14(VINP_FlashOVCL_sec)
  From125/1 -> 0xF88E - 0xF890/15(VDID_FlashAvgBattTempOVCL_C)
  From129/1 -> 0xF88E - 0xF890/16(VINP_FlashOFFR_sec)
  From131/1 -> 0xF88E - 0xF890/17(VDID_FlashAvgBattTempOFFR_C)
  From132/1 -> 0xF88E - 0xF890/18(VINP_FlashOFFL_sec)
  From133/1 -> 0xF88E - 0xF890/19(VDID_FlashAvgBattTempOFFL_C)
  0xF88E - 0xF890/2(VDID_AvgBattTempPSAL_C) -> Goto75/1
  0xF88E - 0xF890/3(VDID_AvgBattTempOVCR_C) -> Goto76/1
  0xF88E - 0xF890/1(VDID_AvgBattTempPSAR_C) -> Goto74/1
  0xF88E - 0xF890/4(VDID_AvgBattTempOVCL_C) -> Goto77/1
  0xF88E - 0xF890/5(VDID_AvgBattTempOFFR_C) -> Goto78/1
  0xF88E - 0xF890/6(VDID_AvgBattTempOFFL_C) -> Goto79/1
  VINP_FlashCPSAL_sec/1 -> [VINP_FlashCPSAL_sec]
  VINP_FlashCPSAR_sec/1 -> [VINP_FlashCPSAR_sec]
  VINP_FlashPSAL_sec/1 -> [VINP_FlashPSAL_sec]
  VINP_FlashIPSAR_sec/1 -> [VINP_FlashIPSAR_sec]
  VINP_FlashIPSAL_sec/1 -> [VINP_FlashIPSAL_sec]
  VINP_FlashPSAR_sec/1 -> [VINP_FlashPSAR_sec]
  VINP_FlashMILDIST_km/1 -> [VINP_FlashMILDIST_km]
  VINP_FlashWARMUPS_cnt/1 -> [VINP_FlashWARMUPS_cnt]
  VINP_FlashDelayCLRDIST_km/1 -> [VINP_FlashDelayCLRDIST_km]
  VINP_FlashMILTime_min/1 -> [VINP_FlashMILTime_min]
  VINP_FlashCLRTime_min/1 -> [VINP_FlashCLRTime_min]
  VINP_FlashNUMPSATRIPSFLTMEMCLR_cnt/1 -> [VINP_FlashNUMPSATRIPSFLTMEMCLR_cnt]
  VINP_FlashTNBCPSAL_Ahr/1 -> [VINP_FlashTNBCPSAL_Ahr]
  VINP_CANMsgValidBMS6_flg/1 -> [VINP_CANMsgValidBMS6_flg]
  VINP_FlashTEBPSAL_kWh/1 -> [VINP_FlashTEBPSAL_kWh]
  VINP_FlashTNECPSAR_kWh/1 -> [VINP_FlashTNECPSAR_kWh]
  VINP_FlashGECHGOVCACR_kWh/1 -> [VINP_FlashGECHGOVCACR_kWh]
  VINP_FlashTGEOVCL_kWh/1 -> [VINP_FlashTGEOVCL_kWh]
  VINP_FlashTGEOVCR_kWh/1 -> [VINP_FlashTGEOVCR_kWh]
  VINP_FlashGECHGOVCACL_kWh/1 -> [VINP_FlashGECHGOVCACL_kWh]
  VINP_FlashTEBPSAR_kWh/1 -> [VINP_FlashTEBPSAR_kWh]
  VINP_FlashGECHGOVCDCR_kWh/1 -> [VINP_FlashGECHGOVCDCR_kWh]
  VINP_FlashTNBCPSAR_Ahr/1 -> [VINP_FlashTNBCPSAR_Ahr]
  VINP_FlashRESSV2XENNONPSAL_kWh/1 -> [VINP_FlashRESSV2XENNONPSAL_kWh]
  VINP_FlashRESSV2XENNONPSAR_kWh/1 -> [VINP_FlashRESSV2XENNONPSAR_kWh]
  VINP_FlashTNECPSAL_kWh/1 -> [VINP_FlashTNECPSAL_kWh]
  VINP_FlashGECHGOVCDCL_kWh/1 -> [VINP_FlashGECHGOVCDCL_kWh]
  VINP_FlashIGNCNTR_cnt/1 -> [VINP_FlashIGNCNTR_cnt]
  VINP_FlashHVBNAH_Ah/1 -> [VINP_FlashHVBNAH_Ah]
  Unit Delay5/1 -> Initial Value4/2
  Initial Value4/1 -> Switch9/3
  [VINP_FlashODOMETER_km] -> Initial Value4/1
  VINP_FlashODOMETER_km/1 -> [VINP_FlashODOMETER_km]
  VINP_FlashPKERNumerator_kphsqr/1 -> [VINP_FlashPKERNumerator_kphsqr]
  VINP_FlashPKELNumerator_kphsqr/1 -> [VINP_FlashPKELNumerator_kphsqr]
  VINP_FlashResetCDEODTR_km/1 -> [VINP_FlashResetCDEODTR_km]
  VINP_FlashAvgBattTempOVCL_C/1 -> [VINP_FlashAvgBattTempOVCL_C]
  VINP_FlashOVCR_sec/1 -> [VINP_FlashOVCR_sec]
  VINP_FlashAvgBattTempPSAL_C/1 -> [VINP_FlashAvgBattTempPSAL_C]
  VINP_FlashTempPSAL_sec/1 -> [VINP_FlashTempPSAL_sec]
  VINP_FlashAvgBattTempOFFL_C/1 -> [VINP_FlashAvgBattTempOFFL_C]
  VINP_FlashAvgBattTempPSAR_C/1 -> [VINP_FlashAvgBattTempPSAR_C]
  VINP_FlashAvgBattTempOFFR_C/1 -> [VINP_FlashAvgBattTempOFFR_C]
  VINP_FlashTempPSAR_sec/1 -> [VINP_FlashTempPSAR_sec]
  VINP_FlashOVCL_sec/1 -> [VINP_FlashOVCL_sec]
  VINP_FlashOFFL_sec/1 -> [VINP_FlashOFFL_sec]
  VINP_FlashOFFR_sec/1 -> [VINP_FlashOFFR_sec]
  VINP_FlashAvgBattTempOVCR_C/1 -> [VINP_FlashAvgBattTempOVCR_C]
  Data Type Conversion7/1 -> Goto138/1
  [VDID_VSS_kph] -> VDID_VSS_kph/1  "VDID_VSS_kph"
  [VDID_RUNTM_s] -> VDID_RUNTM_s/1  "VDID_RUNTM_s"
  [VDID_MILDIST_km] -> VDID_MILDIST_km/1  "VDID_MILDIST_km"
  [VDID_CLRDIST_km] -> VDID_CLRDIST_km/1  "VDID_CLRDIST_km"
  [VDID_APPD_pct] -> VDID_APPD_pct/1  "VDID_APPD_pct"
  [VDID_APPE_pct] -> VDID_APPE_pct/1  "VDID_APPE_pct"
  [VDID_ODOMETER_km] -> VDID_ODOMETER_km/1  "VDID_ODOMETER_km"
  [VDID_NUMPSATRIPSFLTMEMCLR_cnt] -> VDID_NUMPSATRIPSFLTMEMCLR_cnt/1  "VDID_NUMPSATRIPSFLTMEMCLR_cnt"
  [VDID_CPSAL_sec] -> VDID_CPSAL_sec/1  "VDID_CPSAL_sec"
  [VDID_CPSAR_sec] -> VDID_CPSAR_sec/1  "VDID_CPSAR_sec"
  [VDID_PSAR_sec] -> VDID_PSAR_sec/1  "VDID_PSAR_sec"
  [VDID_PSAL_sec] -> VDID_PSAL_sec/1  "VDID_PSAL_sec"
  [VDID_IPSAR_sec] -> VDID_IPSAR_sec/1  "VDID_IPSAR_sec"
  [VDID_IPSAL_sec] -> VDID_IPSAL_sec/1  "VDID_IPSAL_sec"
  Gain20/1 -> Goto99/1
  Gain14/1 -> Goto103/1
  [VDID_PKER_kphsqr] -> VDID_PKER_kphsqr/1  "VDID_PKER_kphsqr"
  [VDID_PKEL_kphsqr] -> VDID_PKEL_kphsqr/1  "VDID_PKEL_kphsqr"
  [VDID_ResetCDEODTR_km] -> VDID_ResetCDEODTR_km/1  "VDID_ResetCDEODTR_km"
  [VDID_CDEODTR_km] -> VDID_CDEODTR_km/1  "VDID_CDEODTR_km"
  [VDID_CDEODTL_km] -> VDID_CDEODTL_km/1  "VDID_CDEODTL_km"
  VINP_FlashHVBNE_kWh/1 -> [VINP_FlashHVBNE_kWh]
  VINP_CANMsgValidBMS1_flg/1 -> [VINP_CANMsgValidBMS1_flg]
  VINP_CANMsgValidCCU2_flg/1 -> [VINP_CANMsgValidCCU2_flg]
  VINP_CANMsgValidBMS4_flg/1 -> [VINP_CANMsgValidBMS4_flg]
  VINP_CellTempAvg_C/1 -> [VINP_CellTempAvg_C]
  Data Type Conversion13/1 -> [VDID_CDEODTL_km]
  [VINP_CANMsgValidMETER1_flg] -> Logical Operator1/2
  Subtract1/1 -> Add2/2
  Max1/1 -> Unit Delay4/1, [VDID_CLRDIST_km]
  Constant17/1 -> Data Type Conversion3/1
  Data Type Conversion3/1 -> Max1/2
  Constant4/1 -> Data Type Conversion2/1
  Data Type Conversion2/1 -> Max/2
  Saturation/1 -> [VDID_APPD_pct]
  From208/1 -> Logical Operator7/2
  NOT2/1 -> Logical Operator7/1
  Logical Operator7/1 -> Minutes_Counter/2
  Unit Delay7/1 -> [VDID_DelayNUMPSATRIPSFLTMEMCLR_cnt]
  Switch6/1 -> Switch5/3
  Switch5/1 -> Unit Delay7/1, [VDID_NUMPSATRIPSFLTMEMCLR_cnt]
  Initial Value5/1 -> Switch6/3
  [VDID_DelayNUMPSATRIPSFLTMEMCLR_cnt] -> Initial Value5/2
  [VINP_FlashNUMPSATRIPSFLTMEMCLR_cnt] -> Initial Value5/1
  [VINP_FlashNUMPSATRIPSFLTMEMCLR_cnt] -> Initial Value6/1
  [VDID_DelayNUMPSATRIPSFLTMEMCLR_cnt] -> Initial Value6/2
  Initial Value6/1 -> Add3/1
  VINP_OBCV2LSta_enum/1 -> [VINP_OBCV2LSta_enum]
  From222/1 -> 0xF885 - 0xF88B/26(VINP_OBCV2LSta_enum)
  Logical Operator4/1 -> NOT4/1, Timer6/1
  Equal9/1 -> Logical Operator4/1
  NOT3/1 -> Logical Operator4/2
  [VPMM_SysPowerMode_enum] -> Equal13/1
  Constant26/1 -> Equal13/2
  Equal13/1 -> Detect Increase1/1
  Detect Increase1/1 -> Initializable_U32counter/1
  Initializable_U32counter/1 -> [VDID_QTYPSATRIPSR_cnt]
  Constant33/1 -> Initializable_U32counter/3
  [VDID_NoteAResetCondition_flg] -> Initializable_U32counter/2
  [VINP_FlashQTYPSATRIPSR_cnt] -> Initializable_U32counter/4
  [VINP_FlashQTYPSATRIPSL_cnt] -> Initializable_U32counter1/4
  Constant35/1 -> Initializable_U32counter1/3
  Initializable_U32counter1/1 -> [VDID_QTYPSATRIPSL_cnt]
  Detect Increase3/1 -> Initializable_U32counter1/1
  Equal15/1 -> Detect Increase3/1
  Constant34/1 -> Equal15/2
  [VPMM_SysPowerMode_enum] -> Equal15/1
  Ground/1 -> Initializable_U32counter1/2
  VINP_FlashQTYPSATRIPSR_cnt/1 -> [VINP_FlashQTYPSATRIPSR_cnt]
  VINP_FlashQTYPSATRIPSL_cnt/1 -> [VINP_FlashQTYPSATRIPSL_cnt]
  [VDID_QTYPSATRIPSR_cnt] -> VDID_QTYPSATRIPSR_cnt/1  "VDID_QTYPSATRIPSR_cnt"
  [VDID_QTYPSATRIPSL_cnt] -> VDID_QTYPSATRIPSL_cnt/1  "VDID_QTYPSATRIPSL_cnt"
  0xF898-0xF8/1(VDID_RESSCNTDODRNGR_cnt) -> Goto153/1
  0xF898-0xF8/15(VDID_AVGBATTEMPL_C) -> Goto167/1
  0xF898-0xF8/14(VDID_MINBATTEMPL_C) -> Goto166/1
  0xF898-0xF8/13(VDID_MAXBATTEMPL_C) -> Goto165/1
  0xF898-0xF8/12(VDID_RESSTIMESOCOFFRNGL_s) -> Goto164/1
  0xF898-0xF8/11(VDID_RESSTIMESOCOFFRNGR_s) -> Goto163/1
  0xF898-0xF8/10(VDID_RESSTIMESOCCHGRNGL_s) -> Goto162/1
  0xF898-0xF8/9(VDID_RESSTIMESOCCHGRNGR_s) -> Goto161/1
  0xF898-0xF8/8(VDID_RESSTIMESOCPSARNGL_s) -> Goto160/1
  0xF898-0xF8/7(VDID_RESSTIMESOCPSARNGR_s) -> Goto159/1
  0xF898-0xF8/6(VDID_ETMBTOEL_kWh) -> Goto158/1
  0xF898-0xF8/5(VDID_ETMBTOER_kWh) -> Goto157/1
  0xF898-0xF8/4(VDID_ETMATOEL_kWh) -> Goto156/1
  0xF898-0xF8/3(VDID_ETMATOER_kWh) -> Goto155/1
  0xF898-0xF8/2(VDID_RESSCNTDODRNGL_cnt) -> Goto154/1
  From245/1 -> 0xF898-0xF8/1(VDID_HVBattPwr_kW)
  From248/1 -> 0xF898-0xF8/4(VDID_NoteAResetCondition_flg)
  From249/1 -> 0xF898-0xF8/5(VINP_FlashRESSCNTDODRNGR_cnt)
  From246/1 -> 0xF898-0xF8/2(task_time_s)
  From247/1 -> 0xF898-0xF8/3(VINP_CANMsgValidBMS1_flg)
  From250/1 -> 0xF898-0xF8/6(VINP_FlashRESSCNTDODRNGL_cnt)
  From254/1 -> 0xF898-0xF8/10(VINP_FlashETMATOEL_kWh)
  From251/1 -> 0xF898-0xF8/7(VINP_RrMCUDCBusCurr_A)
  From252/1 -> 0xF898-0xF8/8(VINP_RrMCUDCBusVolt_V)
  From253/1 -> 0xF898-0xF8/9(VINP_FlashETMATOER_kWh)
  From255/1 -> 0xF898-0xF8/11(VINP_CANMsgValidMCUBR1_flg)
  From256/1 -> 0xF898-0xF8/12(VINP_FrMCUDCBusCurr_A)
  From257/1 -> 0xF898-0xF8/13(VINP_FrMCUDCBusVolt_V)
  From258/1 -> 0xF898-0xF8/14(VINP_FlashETMBTOER_kWh)
  From259/1 -> 0xF898-0xF8/15(VINP_FlashETMBTOEL_kWh)
  From265/1 -> 0xF898-0xF8/21(VINP_FlashRESSTIMESOCPSARNGR_s)
  From260/1 -> 0xF898-0xF8/16(VINP_CANMsgValidMCUBF1_flg)
  From264/1 -> 0xF898-0xF8/20(VINP_HVBattSOC_pct)
  From261/1 -> 0xF898-0xF8/17(VPMM_SysPowerMode_enum)
  From266/1 -> 0xF898-0xF8/22(VINP_FlashRESSTIMESOCPSARNGL_s)
  From262/1 -> 0xF898-0xF8/18(VINP_ChrgPlugSta_enum)
  From267/1 -> 0xF898-0xF8/23(VINP_ExtChrgSta_enum)
  From263/1 -> 0xF898-0xF8/19(VINP_CANMsgValidBMS6_flg)
  From268/1 -> 0xF898-0xF8/24(VINP_FlashRESSTIMESOCCHGRNGR_s)
  From269/1 -> 0xF898-0xF8/25(VINP_FlashRESSTIMESOCCHGRNGL_s)
  From275/1 -> 0xF898-0xF8/28(VDID_FlashMAXBATTEMPL_C)
  From271/1 -> 0xF898-0xF8/27(VINP_FlashRESSTIMESOCOFFRNGL_s)
  From276/1 -> 0xF898-0xF8/29(VINP_HVBMTempMax_C)
  From270/1 -> 0xF898-0xF8/26(VINP_FlashRESSTIMESOCOFFRNGR_s)
  From277/1 -> 0xF898-0xF8/30(VINP_CANMsgValidMETER1_flg)
  From279/1 -> 0xF898-0xF8/32(VINP_HVBMTempMin_C)
  From278/1 -> 0xF898-0xF8/31(VDID_FlashMINBATTEMPL_C)
  From281/1 -> 0xF898-0xF8/34(VINP_FlashAVGBATTEMPL_sec)
  From280/1 -> 0xF898-0xF8/33(VINP_CANMsgValidBMS4_flg)
  From282/1 -> 0xF898-0xF8/35(VDID_FlashAVGBATTEMPL_C)
  From283/1 -> 0xF898-0xF8/36(VINP_CellTempAvg_C)
  VINP_FlashRESSCNTDODRNGR_cnt/1 -> [VINP_FlashRESSCNTDODRNGR_cnt]
  VINP_FlashRESSCNTDODRNGL_cnt/1 -> [VINP_FlashRESSCNTDODRNGL_cnt]
  VINP_RrMCUDCBusCurr_A/1 -> [VINP_RrMCUDCBusCurr_A]
  VINP_RrMCUDCBusVolt_V/1 -> [VINP_RrMCUDCBusVolt_V]
  VINP_FlashETMATOER_kWh/1 -> [VINP_FlashETMATOER_kWh]
  VINP_FlashETMATOEL_kWh/1 -> [VINP_FlashETMATOEL_kWh]
  VINP_FlashAVGBATTEMPL_C/1 -> [VINP_FlashAVGBATTEMPL_C]
  VINP_FlashAVGBATTEMPL_sec/1 -> [VINP_FlashAVGBATTEMPL_sec]
  VINP_FlashMINBATTEMPL_C/1 -> [VINP_FlashMINBATTEMPL_C]
  VINP_HVBMTempMax_C/1 -> [VINP_HVBMTempMax_C]
  VINP_HVBMTempMin_C/1 -> [VINP_HVBMTempMin_C]
  VINP_FlashMAXBATTEMPL_C/1 -> [VINP_FlashMAXBATTEMPL_C]
  VINP_FlashRESSTIMESOCOFFRNGL_s/1 -> [VINP_FlashRESSTIMESOCOFFRNGL_s]
  VINP_FlashRESSTIMESOCOFFRNGR_s/1 -> [VINP_FlashRESSTIMESOCOFFRNGR_s]
  VINP_FlashRESSTIMESOCCHGRNGL_s/1 -> [VINP_FlashRESSTIMESOCCHGRNGL_s]
  VINP_FlashRESSTIMESOCCHGRNGR_s/1 -> [VINP_FlashRESSTIMESOCCHGRNGR_s]
  VINP_FlashRESSTIMESOCPSARNGL_s/1 -> [VINP_FlashRESSTIMESOCPSARNGL_s]
  VINP_FlashRESSTIMESOCPSARNGR_s/1 -> [VINP_FlashRESSTIMESOCPSARNGR_s]
  VINP_CANMsgValidMCUBF1_flg/1 -> [VINP_CANMsgValidMCUBF1_flg]
  VINP_FlashETMBTOEL_kWh/1 -> [VINP_FlashETMBTOEL_kWh]
  VINP_FlashETMBTOER_kWh/1 -> [VINP_FlashETMBTOER_kWh]
  VINP_FrMCUDCBusVolt_V/1 -> [VINP_FrMCUDCBusVolt_V]
  VINP_FrMCUDCBusCurr_A/1 -> [VINP_FrMCUDCBusCurr_A]
  Constant36/1 -> Data Type Conversion4/1
  [VDID_PROTOCOLID_enum] -> VDID_PRO TOCOLID_enum/1  "VDID_PROTOCOLID_enum"
  Data Type Conversion4/1 -> [VDID_PROTOCOLID_enum]
  From285/1 -> 0xF898-0xF8/37(VDID_HVBattPwrDischrg_kW)
  VINP_CANMsgValidBMS3_flg/1 -> [VINP_CANMsgValidBMS3_flg]
  VINP_MCUBFRealPwrKwSta_kW/1 -> [VINP_MCUBFRealPwrKwSta_kW]
  VINP_MCUBRRealPwrKwSta_kW/1 -> [VINP_MCUBRRealPwrKwSta_kW]
  From286/1 -> 0xF898-0xF8/38(VINP_MCUBRRealPwrKwSta_kW)
  From287/1 -> 0xF898-0xF8/39(VINP_MCUBFRealPwrKwSta_kW)
  From288/1 -> 0xF898-0xF8/40(VINP_CANMsgValidBMS3_flg)
  0xF898-0xF8/16(VDID_RESSTTEMPRNGAXIS_enum) -> Goto176/1
  0xF898-0xF8/17(VDID_RESSTIMESOCRNGAXIS_enum) -> Goto182/1
  0xF898-0xF8/18(VDID_RESSCNTSDODRNGAXIS_enum) -> Goto183/1
  String to ASCII2/1 -> Mux/3
  String Constant2/1 -> String to ASCII2/1
  String Constant/1 -> String to ASCII/1
  String to ASCII1/1 -> Mux/2
  String Constant1/1 -> String to ASCII1/1
  String to ASCII/1 -> Mux/1
  VINP_VehicleType_enum/1 -> [VINP_VehicleType_enum]
  VINP_CarModel1_cnt/1 -> [VINP_CarModel1_cnt]
  VINP_CarModel2_cnt/1 -> [VINP_CarModel2_cnt]
  VINP_ECU2_cnt/1 -> [VINP_ECU2_cnt]
  VINP_ECU1_cnt/1 -> [VINP_ECU1_cnt]
  VINP_CarModel3_cnt/1 -> [VINP_CarModel3_cnt]
  VINP_Major1_cnt/1 -> [VINP_Major1_cnt]
  VINP_Major2_cnt/1 -> [VINP_Major2_cnt]
  VINP_Minor1_cnt/1 -> [VINP_Minor1_cnt]
  VINP_ECUGen2_cnt/1 -> [VINP_ECUGen2_cnt]
  VINP_ECUGen1_cnt/1 -> [VINP_ECUGen1_cnt]
  VINP_Variation_cnt/1 -> [VINP_Variation_cnt]
  VINP_Patch2_cnt/1 -> [VINP_Patch2_cnt]
  VINP_Country1_cnt/1 -> [VINP_Country1_cnt]
  VINP_Country2_cnt/1 -> [VINP_Country2_cnt]
  VINP_Patch1_cnt/1 -> [VINP_Patch1_cnt]
  VINP_Minor2_cnt/1 -> [VINP_Minor2_cnt]
  [VINP_CarModel3_cnt] -> Mux1/3
  [VINP_CarModel2_cnt] -> Mux1/2
  [VINP_CarModel1_cnt] -> Mux1/1
  [VDID_CALID_cnt] -> VDID_CALID_cnt/1  "VDID_CALID_cnt"
  [VDID_ECUNAME_cnt] -> VDID_ECUNAME_cnt/1  "VDID_ECUNAME_cnt"
  [VDID_PKERNumerator_kphsqr] -> VDID_PKERNumerator_kphsqr/1  "VDID_PKERNumerator_kphsqr"
  [VDID_PKELNumerator_kphsqr] -> VDID_PKELNumerator_kphsqr/1  "VDID_PKELNumerator_kphsqr"
  0xF898-0xF8/19(VDID_AVGBATTEMPL_sec) -> Goto215/1
  0xF88E - 0xF890/7(VDID_BattTempPSAR_sec) -> Goto216/1
  0xF88E - 0xF890/8(VDID_BattTempPSAL_sec) -> Goto217/1
  0xF88E - 0xF890/9(VDID_OVCR_sec) -> Goto218/1
  0xF88E - 0xF890/10(VDID_OVCL_sec) -> Goto219/1
  0xF88E - 0xF890/11(VDID_OFFR_sec) -> Goto220/1
  0xF88E - 0xF890/12(VDID_OFFL_sec) -> Goto221/1
  Mux1/1 -> Data Type Conversion5/1
  Data Type Conversion5/1 -> [VDID_CALID_cnt]
  Mux/1 -> Data Type Conversion11/1
  [VINP_Major1_cnt] -> Mux1/4
  [VINP_Major2_cnt] -> Mux1/5
  [VINP_Minor1_cnt] -> Mux1/6
  [VINP_Minor2_cnt] -> Mux1/7
  [VINP_Patch1_cnt] -> Mux1/8
  [VINP_Patch2_cnt] -> Mux1/9
  [VINP_Country1_cnt] -> Mux1/10
  [VINP_Country2_cnt] -> Mux1/11
  [VINP_Variation_cnt] -> Mux1/12
  [VINP_ECUGen1_cnt] -> Mux1/13
  [VINP_ECUGen2_cnt] -> Mux1/14
  VPMM_DrivetrainSelect_enum/1 -> [VPMM_DrivetrainSelect_enum]
  [VDID_DrivingMode_cnt] -> Mux1/15
  [VPMM_DrivetrainSelect_enum] -> 1-D Lookup Table/1
  [VPMM_DrivetrainSelect_enum] -> Equal16/1
  Constant39/1 -> Equal16/2
  Constant40/1 -> Equal17/2
  [VPMM_DrivetrainSelect_enum] -> Equal17/1
  [VPMM_DrivetrainSelect_enum] -> Equal21/1
  Constant41/1 -> Equal21/2
  Equal16/1 -> OR/1
  Equal17/1 -> OR/2
  Equal21/1 -> OR/3
  OR/1 -> Switch7/2
  1-D Lookup Table/1 -> Switch7/1
  Switch7/1 -> [VDID_DrivingMode_cnt]
  String to ASCII3/1 -> Switch7/3
  String Constant3/1 -> String to ASCII3/1
  [VDID_ModelYear_cnt] -> Mux1/16
  String Constant4/1 -> String to ASCII4/1
  String to ASCII4/1 -> [VDID_ModelYear_cnt]
  VINP_VinCode_cnt/1 -> [VINP_VinCode_cnt]
  [VINP_VinCode_cnt] -> Data Type Conversion14/1
  Data Type Conversion14/1 -> [VDID_VinCode_cnt]
  [VDID_VinCode_cnt] -> VDID_VinCode_cnt/1  "VDID_VinCode_cnt"
  [VDID_DelayCLRDIST_km] -> Add2/1
  Initial Value/1 -> Switch4/3
  Add2/1 -> Initial Value/2
  [VINP_FlashDelayCLRDIST_km] -> Initial Value/1
  Constant45/1 -> Shift Arithmetic313/1
  Shift Arithmetic313/1 -> Bitwise OR123/4
  Constant44/1 -> Shift Arithmetic312/1
  Constant42/1 -> Bitwise OR123/1
  Shift Arithmetic312/1 -> Bitwise OR123/3
  Constant43/1 -> Shift Arithmetic311/1
  Shift Arithmetic311/1 -> Bitwise OR123/2
  Shift Arithmetic1/1 -> Bitwise OR123/5
  Shift Arithmetic2/1 -> Bitwise OR123/6
  Shift Arithmetic3/1 -> Bitwise OR123/7
  Shift Arithmetic4/1 -> Bitwise OR123/8
  Constant47/1 -> Shift Arithmetic1/1
  Constant48/1 -> Shift Arithmetic2/1
  Constant51/1 -> Shift Arithmetic3/1
  Constant52/1 -> Shift Arithmetic4/1
  Constant63/1 -> Shift Arithmetic11/1
  Constant62/1 -> Shift Arithmetic7/1
  Constant61/1 -> Shift Arithmetic6/1
  Constant58/1 -> Shift Arithmetic5/1
  Shift Arithmetic8/1 -> Bitwise OR1/2
  Constant53/1 -> Bitwise OR1/1
  Constant57/1 -> Shift Arithmetic10/1
  Shift Arithmetic11/1 -> Bitwise OR1/7
  Shift Arithmetic7/1 -> Bitwise OR1/6
  Shift Arithmetic6/1 -> Bitwise OR1/5
  Shift Arithmetic5/1 -> Bitwise OR1/4
  Shift Arithmetic10/1 -> Bitwise OR1/3
  Data Type Conversion15/1 -> Goto227/1
  From325/1 -> Data Type Conversion15/1
  Bitwise OR1/1 -> Data Type Conversion17/1
  Bitwise OR123/1 -> Data Type Conversion16/1
  Constant54/1 -> Shift Arithmetic8/1
  Data Type Conversion16/1 -> Goto229/1
  Data Type Conversion17/1 -> Goto228/1
  Data Type Conversion11/1 -> Reshape/1
  Reshape/1 -> [VDID_ECUNAME_cnt]
  Add/1 -> Initial Value2/2
  Initial Value2/1 -> Switch/1
  NOT4/1 -> Timer6/2
  Subsystem/1(VDID_DIDModelVersion_raw) -> [VDID_DIDModelVersion_raw]
  Cast To Boolean/1 -> Subsystem/Enable
  Subsystem/2(VDID_DIDModelVersionChksum_raw) -> [VDID_DIDModelVersionChksum_raw]
  Constant64/1 -> Delay1/1
  Logical Operator8/1 -> Cast To Boolean/1
  Delay1/1 -> Logical Operator8/1
  VINP_FlashModelVersion_raw/1 -> [VINP_FlashModelVersion_raw]
  VINP_FlashModelVersionChksum_raw/1 -> [VINP_FlashModelVersionChksum_raw]
  [VINP_FlashModelVersion_raw] -> Checksum/1(ModelVersion)
  [VINP_FlashModelVersionChksum_raw] -> Equal22/2
  Constant55/1 -> Equal23/2
  [VDID_DIDModelVersion_raw] -> Equal23/1
  Equal23/1 -> Logical Operator9/1
  Checksum/1(ModelVersionChksum) -> Equal22/1
  Equal22/1 -> [VDID_ModelVersionChksumValid_flg]
  [VDID_ModelVersionChksumValid_flg] -> Logical Operator9/2
  Logical Operator9/1 -> [VDID_FlashValid_flg]
  [VDID_DIDModelVersionChksum_raw] -> VDID_DIDModelVersionChksum_raw/1  "VDID_DIDModelVersionChksum_raw"
  [VDID_DIDModelVersion_raw] -> VDID_DIDModelVersion_raw/1  "VDID_DIDModelVersion_raw"
  From336/1 -> Switch14/1
  From335/1 -> Switch14/2
  Constant65/1 -> Switch14/3
  Switch14/1 -> Goto140/1
  Switch15/1 -> Goto237/1
  Constant68/1 -> Switch15/3
  From337/1 -> Switch15/2
  From338/1 -> Switch15/1
  From339/1 -> Switch17/2
  Constant69/1 -> Switch17/3
  Constant72/1 -> Switch20/3
  From345/1 -> Switch20/2
  From343/1 -> Switch19/2
  Constant71/1 -> Switch19/3
  Constant70/1 -> Switch18/3
  From341/1 -> Switch18/2
  Constant73/1 -> Switch23/3
  From340/1 -> Switch23/2
  From342/1 -> Switch24/2
  Constant74/1 -> Switch24/3
  From349/1 -> Switch17/1
  From344/1 -> Switch18/1
  From346/1 -> Switch19/1
  From347/1 -> Switch20/1
  From348/1 -> Switch23/1
  From350/1 -> Switch24/1
  Switch17/1 -> Goto238/1
  Switch18/1 -> Goto239/1
  Switch19/1 -> Goto240/1
  Switch20/1 -> Goto241/1
  Switch23/1 -> Goto242/1
  Switch24/1 -> Goto243/1
  Constant75/1 -> Switch25/3
  From354/1 -> Switch25/2
  From351/1 -> Switch25/1
  From355/1 -> Switch26/2
  Constant76/1 -> Switch26/3
  From352/1 -> Switch26/1
  Constant77/1 -> Switch27/3
  From356/1 -> Switch27/2
  From353/1 -> Switch27/1
  Switch25/1 -> Goto244/1
  Switch26/1 -> Goto245/1
  Switch27/1 -> Goto246/1
  Latch2/1 -> Unit Delay8/1
  Unit Delay9/1 -> Initial Value9/2
  From379/1 -> Detect Increase4/1
  From369/1 -> Minus3/2
  Minus4/1 -> Switch31/1
  Unit Delay8/1 -> Switch28/2
  Unit Delay3/1 -> Switch28/1
  Detect Increase4/1 -> Latch2/1
  From378/1 -> Minus4/2
  Switch28/1 -> Unit Delay3/1, Goto251/1
  From371/1 -> Switch29/1
  From374/1 -> Minus7/1
  From368/1 -> Minus3/1
  From370/1 -> Detect Decrease/1
  From376/1 -> Switch30/3
  From377/1 -> Minus5/2
  Detect Decrease/1 -> Switch29/2
  Minus7/1 -> Switch30/1
  Switch29/1 -> Goto247/1, Unit Delay9/1
  Switch31/1 -> Minus5/1, Unit Delay10/1
  From380/1 -> Switch31/2
  From381/1 -> Minus4/1
  Initial Value9/1 -> Switch29/3
  Minus5/1 -> Goto250/1
  Unit Delay10/1 -> Initial Value10/2
  From367/1 -> Initial Value10/1
  From373/1 -> Minus6/1
  Detect Increase5/1 -> Switch30/2
  Delay2/1 -> Goto249/1
  From372/1 -> Minus6/2
  From375/1 -> Detect Increase5/1
  Switch30/1 -> Delay2/1, Goto248/1
  Initial Value10/1 -> Switch31/3
  From357/1 -> Initial Value9/1
  Minus6/1 -> Minus7/2
  Minus3/1 -> Switch28/3
